simulink library "DAEMOT_Lib"  (R2019b)
settings: Solver=ode45  StartTime=0.0  StopTime=10.0  FixedStep=0.1  RelTol=1e-3
undefined symbols (not defined in the file or in its folder): Controller, CP, Ctrl, Ctrl_Fcn, Elec1, f, F2, Fluid, lag1, Mission, Moody, PropellerProp, rev_comms_sink
libraries: $bdroot x200, instrumentlib x21, simulink x5, dspsigops x2
(part 3 of 13)

== system DAEMOT_Lib/Legacy Components ==
  Aircraft : Subsystem  mask(Fluid Tank){Vel_init=300, M_dry=108500, M_load=21337, rho=0.243, A=360, Cd=0.02439}
      mask prompts: Vel_init "Initial Velocity [m/s]"; M_dry "Dry Weight [kg]"; M_load "Payload Weight [kg]"; rho "Air Density [kg/m^3]"; A "Reference Area [m²]"; Cd "Drag Coefficient [-]"
      mask help: Tracks the time rate of change for fluid mass and temperature.
      settings: OpenFcn=|
      | load('Fluids.mat');
      | Set_Fluid_Popup_Names( Fluid )
      mask DialogControl Container8 Prompt: Parameters
      mask Display:
      | image(imread('aircraft.jpg'))
      | 
      | text(0.5,0.9,['{\bf Aircraft}'],'TexMode','on','horizontalAlignment', 'center')
      | 
      | port_label('input',1,'Fuel Mass [kg]')
      | port_label('output',1,'Right Engine')
      | port_label('output',2,'Left Engine')
  Battery : Subsystem  mask{SOC0=0, C=100, P_max=100, T0=20, eta_max=0.98, T_max=100, eta_min=0.8}
      mask prompts: SOC0 "Initial State of Charge [0:1]"; C "Capacitance [MJ]"; P_max "Maximum Power [kW]"; T0 "Maximum Efficiency Temperature [oC]"; eta_max "Maximum Efficiency [0:1]"; T_max "Maximum Temperature [oC]"; eta_min "Minimum Efficiency [0:1]"
      mask init:
      | a = -(eta_max-eta_min)/(T_max-T0)^2;
      | b = -2*a*T0;
      | c = eta_max + a*T0^2;
      mask Display:
      | % text(0.5,0.9,['{\bf Load}'],'TexMode','on','horizontalAlignment', 'center')
      | 
      | port_label('input',1,'Power')
      | port_label('input',2,'Usage')
      | port_label('output',1,'Heat')
  Bus : Subsystem  mask(Bus){}
      mask help: This is a bus.
  Bus1 : Subsystem  mask(Bus){Num_Out=2}
      mask prompts: Num_Out "Number of Outputs"
      mask help: This is a bus.
      mask init:
      | h      = get_param(gcb,'handle');   % Get block handle
      | blk    = gcb;
      | hblock = get(h);     % Parse out handles structure
      | 
      | %%%%%%%%%%%%%%%%%%%%%%%%%%%%%% Clear Stuff %%%%%%%%%%%%%%%%%%%%%%%%%%%%%%%%
      | % delete any previous inports and bus selectors
      | for i = str2num(hblock.Num_Out)+1:hblock.Ports(2)
      |     delete_block([blk,'/Out',num2str(i)])
      |     delete_block([blk,'/b',num2str(i)])
      |     delete_block([blk,'/Source',num2str(i)])
      |     
      |     delete_unconnected_lines(blk)
      | end
      | %%%%%%%%%%%%%%%%%%%%%%%%%%%%%% Clear Stuff %%%%%%%%%%%%%%%%%%%%%%%%%%%%%%%%
      | 
      | %%%%%%%%%%%%%%%%%%%%%%%%%%%%%% Edit Mux inputs %%%%%%%%%%%%%%%%%%%%%%%%%%%%%%%%
      | 
      | set_param([blk,'/Add'],'Inputs',hblock.Num_Out)
      | 
      | %%%%%%%%%%%%%%%%%%%%%%%%%%%%%% Edit Mux inputs %%%%%%%%%%%%%%%%%%%%%%%%%%%%%%%%
      | 
      | %%%%%%%%%%%%%%%%%%%%%%%%%%%%%% Creat and Place Outputs %%%%%%%%%%%%%%%%%%%%%%%%%%%%%%%%
      | % generate outports, bus selectors, and route lines to each vector concat
      | for i = hblock.Ports(2)+1:str2num(hblock.Num_Out)
      |     
      |     % add blocks
      |     add_block('simulink/Ports & Subsystems/Out1',   [blk,'/Out',num2str(i)],   'Position',[900 i*80-25-180 900+30 i*80-12-180]);         % adding outport
      |     add_block('simulink/Signal Routing/Bus Creator',[blk,'/b',num2str(i)],     'Position',[850 i*80-20+20-218 850+5 i*80-2+20-198]);     % adding bus
      |     add_block('DAEMOT_Lib/Support Functions/Source', [blk,'/Source',num2str(i)],'Position',[400 i*80-205 400+65 i*80-180]);         % adding source
      | 
      |     % set bus number of ports
      |     set_param([blk,'/b',num2str(i)],'Inputs','2')
      |     
      | %     % set goto and from background colors
      | %     set_param([blk,'/t',num2str(i)],'BackgroundColor','cyan')
      | %     set_param([blk,'/m',num2str(i)],'BackgroundColor','cyan')
      | %     set_param([blk,'/p',num2str(i)],'BackgroundColor','cyan')
      | %     set_param([blk,'/g',num2str(i)],'BackgroundColor','cyan')
      | %     set_param([blk,'/mout',num2str(i)],'BackgroundColor','cyan')
      | %     %set_param([blk,'/tout',num2str(i)],'BackgroundColor','cyan')
      |     
      |     % add lines
      |     add_line(blk,['in/1'],['b',num2str(i),'/1'],'AutoRouting','on')
      |     
      |     add_line(blk,['Source',num2str(i),'/1'],['b',num2str(i),'/2'],'AutoRouting','on')
      |     p = get_param([blk,'/Source',num2str(i)],'PortHandles');
      |     l = get_param(p.Outport,'Line');
      |     set_param(l,'Name','I')
      |      
      |     add_line(blk,['b',num2str(i),'/1'],['Out',num2str(i),'/1'],'AutoRouting','on')
      |     add_line(blk,['Source',num2str(i),'/1'],['Add/',num2str(i)],'AutoRouting','on')
      | end
      | %%%%%%%%%%%%%%%%%%%%%%%%%%%%%% Create and Place Outputs %%%%%%%%%%%%%%%%%%%%%%%%%%%%%%%%
      | 
      | % try
      | %     set_param([blk,'/Selector1'],'InputPortWidth',num2str(hblock.Num_Out))
      | %     
      | %     selector_str = '[1 ';
      | %     for i = 2:str2num(hblock.Num_Out)
      | %         selector_str = [selector_str,num2str(i),' '];
      | %     end
      | %     selector_str = [selector_str,']'];
      | %     set_param([blk,'/Selector1'],'IndexParamArray',{selector_str})%num2cell(1:hblock.Num_Out))
      | % catch
      | %     selector_str = '[1 ';
      | %     for i = 2:str2num(hblock.Num_Out)
      | %         selector_str = [selector_str,num2str(i),' '];
      | %     end
      | %     selector_str = [selector_str,']'];
      | %     set_param([blk,'/Selector1'],'IndexParamArray',{selector_str})%num2cell(1:hblock.Num_Out))
      | %     
      | %     set_param([blk,'/Selector1'],'InputPortWidth',num2str(hblock.Num_Out))
      | % end 
      |     
      |     clear h blk hblock
      settings: CopyFcn=|
      | h      = get_param(gcb,'handle');   % Get block handle
      | blk    = gcb;
      | 
      | set_param(blk, 'LinkStatus', 'inactive')
      mask DialogControl ParameterTabVar0 Prompt: Bus Parameters
  Cabin : Subsystem  Commented=on  mask(Air Volume (Cabin)){T_init=0, V=0}
      mask prompts: T_init "Initial Temperature [°C]"; V "Volume [m³]"
      mask help: Tracks the time rate of change for the volume's temperature.
      mask init:
      | load Fluids
      | eval(['Fluid = Fluid.Air;']);
      mask DialogControl Container4 Prompt: Parameters
      mask Display:
      | text(0.5,0.95,['{\bf Air Volume}'],'TexMode','on','horizontalAlignment', 'center')
      | 
      | port_label('input',1,['Flow In'])
      | port_label('input',2,['Heat'])
      | port_label('output',1,['Flow Out'])
  Condenser : Subsystem  Commented=on  mask(Condenser){fld2=Water, T_init=0, C_wall=0, Tw0=0, Q0=0, T0=0, Tin_0=0, Tout_0=0, Qout_0=0, mdot2_0=0, H2_0=0, Tin2_0=0, A2=NaN, Rwc=NaN, Rc_in=NaN, Rc_out=NaN}
      mask prompts: fld2 "Secondary Fluid"; T_init "Initial Wall Temperature [°C]"; C_wall "Wall Capacitance [J/K]"; Tw0 "Condenser Wall Temperature [°C]"; Q0 "Wall Heat Transfer Rate [W]"; T0 "Condensing Temperature [°C]"; Tin_0 "Inlet Temperature [°C]"; Tout_0 "Outlet Temperature [°C]"; Qout_0 "Outlet Heat Transfer Rate [W]"; mdot2_0 "Mass Flow Rate [kg/s]"; H2_0 "Heat Transfer Coefficient [W/m²K]"; Tin2_0 "Fluid Inlet Temperature[°C]"; A2 "Heat Transfer Area [m²]"; Rwc "Condenser Wall Resistance"; Rc_in "Condenser Inlet Resistance"; Rc_out "Condenser Outlet Resistance"
      mask help: Tracks the time rate of change of condenser wall temperature. Calculates the outlet temperature and inlet/outlet heat flow.
      mask init:
      | load Fluids
      | eval(['F2 = Fluid.',get_param(gcb,'fld2'),';']);
      | 
      | 
      | area = -(mdot2_0*F2.cp/H2_0)*log(1-Q0/(mdot2_0*F2.cp*(Tw0 - Tin2_0)));    % m^2
      | 
      | Rwc = (T0 - Tw0) / Q0;
      | Rc_in = (Tin_0 - T0) / (Q0 - Qout_0);
      | Rc_out = (T0 - Tout_0)/(Qout_0);
      | 
      | set_param(gcb,'A2',num2str(area))
      | set_param(gcb,'Rwc',num2str(Rwc))
      | set_param(gcb,'Rc_in',num2str(Rc_in))
      | set_param(gcb,'Rc_out',num2str(Rc_out))
      mask TypeOptions fld2: Water | Fuel | Air
      mask DialogControl Container4 Prompt: Parameters
      mask DialogControl Container5 Prompt: Nonlinear Modeling
      mask DialogControl Container9 Prompt: Component Sizing - Nominal Values
      mask DialogControl Container10 Prompt: Primary Side
      mask DialogControl Container11 Prompt: Secondary Side
      mask DialogControl Container6 Prompt: Linear Model
      mask Display:
      | text(0.5,0.95,['{\bf Condenser}'],'TexMode','on','horizontalAlignment', 'center')
      | 
      | port_label('input',1,'Sink In')
      | port_label('input',2,'From Comp.')
      | port_label('input',3,'Inlet Resistance')
      | port_label('output',2,'To Valve')
      | port_label('output',1,'Sink Out')
  Converter : Subsystem  mask(Fluid Tank){V=230, I0=100, eta_max=0.98, eta_min=0.8}
      mask prompts: V "Converter Voltage [V]"; I0 "Maximum Efficiency Current [A]"; eta_max "Maximum Efficiency [0:1]"; eta_min "Minimum Efficiency [0:1]"
      mask help: Tracks the time rate of change for fluid mass and temperature.
      settings: OpenFcn=|
      | load('Fluids.mat');
      | Set_Fluid_Popup_Names( Fluid )
      mask DialogControl Container9 Prompt: Converter Parameters
      mask Display:
      | % image(imread('inverter.jpg'))
      | 
      | text(0.5,0.9,['{\bf Inverter}'],'TexMode','on','horizontalAlignment', 'center')
      | 
      | port_label('input',1,'In')
      | port_label('output',1,'Out')
      | port_label('output',2,'Heat')
  Dist : Subsystem  mask(Dist){}
      mask help: This is a distribution bus.
  Dist1 : Subsystem  mask{Num_In=2}
      mask prompts: Num_In "Number of Inputs"
      mask init:
      | h      = get_param(gcb,'handle');   % Get block handle
      | blk    = gcb;
      | hblock = get(h);     % Parse out handles structure
      | 
      | %%%%%%%%%%%%%%%%%%%%%%%%%%%%%% Clear Stuff %%%%%%%%%%%%%%%%%%%%%%%%%%%%%%%%
      | % delete any previous inports and bus selectors
      | for i = str2num(hblock.Num_In)+1:hblock.Ports(1)-1
      |     delete_block([blk,'/In',num2str(i)])
      |     delete_block([blk,'/b',num2str(i)])
      |     delete_block([blk,'/term',num2str(i)])
      |     delete_block([blk,'/Sink',num2str(i)])
      |     
      |     delete_unconnected_lines(blk)
      | end
      | if str2num(hblock.Num_In)+1 < hblock.Ports(1)-1
      | try
      | delete_block([blk,'/u'])
      | delete_unconnected_lines(blk)
      | end
      | end
      | %%%%%%%%%%%%%%%%%%%%%%%%%%%%%% Clear Stuff %%%%%%%%%%%%%%%%%%%%%%%%%%%%%%%%
      | 
      | %%%%%%%%%%%%%%%%%%%%%%%%%%%%%% Edit Mux inputs %%%%%%%%%%%%%%%%%%%%%%%%%%%%%%%%
      | set_param([blk,'/Mux'],'Inputs',hblock.Num_In)
      | set_param([blk,'/Demux'],'Outputs',hblock.Num_In)
      | %%%%%%%%%%%%%%%%%%%%%%%%%%%%%% Edit Mux inputs %%%%%%%%%%%%%%%%%%%%%%%%%%%%%%%%
      | 
      | %%%%%%%%%%%%%%%%%%%%%%%%%%%%%% Create and Place Inputs %%%%%%%%%%%%%%%%%%%%%%%%%%%%%%%%
      | % generate inports, bus selectors, and route lines to each vector concat
      | for i = hblock.Ports(1):str2num(hblock.Num_In)
      |     
      |     % add blocks
      |     add_block('simulink/Ports & Subsystems/In1',     [blk,'/In',num2str(i)],    'Position',[220 i*80+308 250 i*80+322]);         % adding inport
      |     add_block([blk,'/b1'],                           [blk,'/b',num2str(i)],    'Position',[295 i*80+275 300 i*80+355]);         % adding bus selector
      |     add_block('simulink/Sinks/Terminator',           [blk,'/term',num2str(i)],  'Position',[350 i*80+325 370 i*80+345]);         % adding terminator
      |     add_block('DAEMOT_Lib/Support Functions/Sink',   [blk,'/Sink',num2str(i)],  'Position',[1020 i*20+439 1085 i*20+461]);         % adding sink
      |     
      |     
      |     % set goto and from background colors
      | %    set_param([blk,'/gm',num2str(i)],'BackgroundColor','yellow')
      | %    set_param([blk,'/gt',num2str(i)],'BackgroundColor','yellow')
      | %    %set_param([blk,'/gp',num2str(i)],'BackgroundColor','yellow')
      | %    set_param([blk,'/min',num2str(i)],'BackgroundColor','yellow')
      | %    set_param([blk,'/tin',num2str(i)],'BackgroundColor','yellow')
      | %    set_param([blk,'/pout',num2str(i)],'BackgroundColor','cyan')
      |     
      |     % add lines
      |     add_line(blk,['In',num2str(i),'/1'], ['b',num2str(i),'/1'],'AutoRouting','on')
      |     add_line(blk,['b',num2str(i),'/1'], ['Mux/',num2str(i)],'AutoRouting','on')
      |     add_line(blk,['b',num2str(i),'/2'], ['term',num2str(i),'/1'],'AutoRouting','on')
      |     add_line(blk,['Demux/',num2str(i)], ['Sink',num2str(i),'/1'],'AutoRouting','on')
      |     
      | end
      | try
      |     add_block('simulink/Ports & Subsystems/In1',     [blk,'/u'],    'Position',[635-50 386+15 635-20 400+15]);         % adding control inport
      |     add_line(blk,['u/1'], ['u_tag/1'],'AutoRouting','on')
      | end
      | %%%%%%%%%%%%%%%%%%%%%%%%%%%%%% Creat and Place Inputs %%%%%%%%%%%%%%%%%%%%%%%%%%%%%%%%
      | 
      | % try
      | %     set_param([blk,'/Selector1'],'InputPortWidth',num2str(hblock.Num_In))
      | %     
      | %     selector_str = '[1 ';
      | %     for i = 2:str2num(hblock.Num_In)
      | %         selector_str = [selector_str,num2str(i),' '];
      | %     end
      | %     selector_str = [selector_str,']'];
      | %     set_param([blk,'/Selector1'],'IndexParamArray',{selector_str})%num2cell(1:hblock.Num_In))
      | % catch
      | %     selector_str = '[1 ';
      | %     for i = 2:str2num(hblock.Num_In)
      | %         selector_str = [selector_str,num2str(i),' '];
      | %     end
      | %     selector_str = [selector_str,']'];
      | %     set_param([blk,'/Selector1'],'IndexParamArray',{selector_str})%num2cell(1:hblock.Num_In))
      | %     
      | %     set_param([blk,'/Selector1'],'InputPortWidth',num2str(hblock.Num_In))
      | % end 
      |     
      |     clear h blk hblock
      settings: CopyFcn=|
      | h      = get_param(gcb,'handle');   % Get block handle
      | blk    = gcb;
      | 
      | set_param(blk, 'LinkStatus', 'inactive')
      mask DialogControl ParameterTabVar0 Prompt: Bus Parameters
  Engine : Subsystem  mask(Fluid Tank){fuel=Fuel, P=3500, Omega_init=1000, J=100, Omega_max=1500, Thrust_max=100000, eta=0.25, alpha=0.15}
      mask prompts: fuel "Fuel Type"; P "Engine Pressure [kPa]"; Omega_init "Initial Shaft Speed [rad/s]"; J "Moment of Inertia [kg m²]"; Omega_max "Maximum Shaft Speed [rad/s]"; Thrust_max "Maximum Thrust [N]"; eta "Engine Efficiency [-]"; alpha "Bearing Heat Gen Coeff. [kW/rad/s]"
      mask help: Tracks the time rate of change for fluid mass and temperature.
      mask init:
      | load('Fluids.mat');
      | Fuel = eval(['Fluid.',fuel]);
      settings: OpenFcn=|
      | load('Fluids.mat');
      | Set_Fluid_Popup_Names( Fluid )
      mask TypeOptions fuel: Fuel | Water | Air | PG50
      mask DialogControl Container9 Prompt: Engine Parameters
      mask Display:
      | image(imread('engine.jpg'))
      | 
      | text(0.5,0.9,['{\bf Engine}'],'TexMode','on','horizontalAlignment', 'center')
      | text(0.5,0.1,['{(P)}'],'TexMode','on','horizontalAlignment', 'center')
      | 
      | port_label('input',1,'Aircraft')
      | port_label('input',2,'Fuel In')
      | port_label('output',1,'Generator')
      | port_label('output',2,'Heat')
  Evaporator : Subsystem  Commented=on  mask(Evaporator){src=Heat Source (Q), fld=Fuel, T_init=0, C_wall=0, Tw0=0, Q0=0, T_evap=0, Tin_0=0, Tout_0=0, H0=0, Qin0=0, Qout0=0, mdot2_0=0, T2in_0=0, H2_0=0, A2=0, Rwe=NaN, Re_in=NaN, Re_out=NaN}
      mask prompts: src "Secondary Side Source"; fld "Fluid Type"; T_init "Initial Wall Temperature [°C]"; C_wall "Wall Capacitance [J/K]"; Tw0 "Evaporator Wall Temperature [°C]"; Q0 "Wall Heat Transfer Rate [W]"; T_evap "Evaporation Temperature [°C]"; Tin_0 "Inlet Temperature [°C]"; Tout_0 "Outlet Temperature [°C]"; H0 "Heat Transfer Coefficient [W/m²K]"; Qin0 "Inlet Heat Transfer Rate [W]"; Qout0 "Outlet Heat Transfer Rate [W]"; mdot2_0 "Mass Flow Rate [kg/s]"; T2in_0 "Inlet Temperature [°C]"; H2_0 "Heat Transfer Coefficient [W/m²K]"; A2 "Evaporator Wall Area [m²]"; Rwe "Evaporator Wall Resistance"; Re_in "Evaporator Inlet Resistance"; Re_out "Evaporator Outlet Resistance"
      mask help: Tracks the time rate of change of evaporator wall temperature. Calculates the outlet temperature and inlet/outlet heat flow.
      mask init:
      | load Fluids
      | eval(['F2 = Fluid.',get_param(gcb,'fld'),';']);
      | 
      | 
      | Rwe = (Tw0 - T_evap) / Q0;
      | Re_in = (Tin_0 - T_evap) / (Qin0);
      | Re_out = (T_evap - Tout_0) / (Qout0);
      | 
      | set_param(gcb,'Rwe',num2str(Rwe))
      | set_param(gcb,'Re_in',num2str(Re_in))
      | set_param(gcb,'Re_out',num2str(Re_out))
      | 
      | area = -((mdot2_0)*F2.cp/(H2_0+eps))*log(1-Q0/(mdot2_0*F2.cp*(T2in_0-Tw0)+eps));    % m^2
      |           
      | set_param(gcb,'A2',num2str(area))
      | 
      | 
      | % choices available in the popup menu
      | choices = {'Fluid Flow (Fluid Bus)','Heat Source (Q)'};
      | % index of the current choice
      | ndex = find(strcmp(get_param(gcb,'src'),choices));
      | 
      | if ndex == 1    % if fluid flow bus is selected
      |     try
      |         delete_line(gcb,'In2/1','Q_load_goto/1')
      |         delete_line(gcb,'In1/1','Tin_Bus/1')
      |         add_line(gcb,'In2/1','Tin_Bus/1')
      |     catch
      |     end
      |     set_param([gcb,'/outgain1'],'Gain','1')
      |     set_param([gcb,'/outgain2'],'Gain','1')
      | else            % if it is a heat source 
      |     try
      |         delete_line(gcb,'In2/1','Tin_Bus/1')
      |         add_line(gcb,'In2/1','Q_load_goto/1')
      |         add_line(gcb,'In1/1','Tin_Bus/1')
      |     catch
      |     end
      |     set_param([gcb,'/outgain1'],'Gain','0')
      |     set_param([gcb,'/outgain2'],'Gain','0')
      | end
      | 
      | clear ndex choices
      mask TypeOptions src: Fluid Flow (Fluid Bus) | Heat Source (Q)
      mask Callback src:
      | % choices available in the popup menu
      | choices = {'Fluid Flow (Fluid Bus)','Heat Source (Q)'};
      | % index of the current choice
      | ndex = find(strcmp(get_param(gcb,'src'),choices));
      | % visibility of parameters in the mask
      | mask_vis = get_param(gcb,'MaskVisibilities');
      | 
      | % maskobj = Simulink.Mask.get(gcb);
      | % dialogobj = maskobj.getDialogControls();
      | % grpobj = dialogobj(1, 2).DialogControls(1, 2).DialogControls.DialogControls(1, 5);
      | 
      | if ndex == 1    % if fluid flow bus is selected
      |     mask_vis{2} = 'on';    mask_vis{13} = 'on';    mask_vis{14} = 'on';
      |     mask_vis{15} = 'on';    mask_vis{16} = 'on';
      | 
      | else            % if it is a heat source
      |     mask_vis{2} = 'off';    mask_vis{13} = 'off';    mask_vis{14} = 'off';
      |     mask_vis{15} = 'off';    mask_vis{16} = 'off';
      | 
      | end
      | 
      | % setting the new visibility
      | set_param(gcb,'MaskVisibilities',mask_vis)
      | 
      | clear ndex choices mask_vis maskobj dialogobj grpobj
      mask TypeOptions fld: Fuel | Water | Air
      mask DialogControl Container4 Prompt: Parameters
      mask DialogControl Container5 Prompt: Nonlinear Model
      mask DialogControl Container7 Prompt: Component Sizing - Nominal Values
      mask DialogControl Container9 Prompt: Primary Side
      mask DialogControl SecSideContainer Prompt: Secondary Side
      mask DialogControl Container6 Prompt: Linear Model
      mask Display:
      | text(0.5,0.95,['{\bf Evaporator}'],'TexMode','on','horizontalAlignment', 'center')
      | 
      | port_label('input',1,'From Valve')
      | % choices available in the popup menu
      | choices = {'Fluid Flow (Fluid Bus)','Heat Source (Q)'};
      | % index of the current choice
      | ndex = find(strcmp(get_param(gcb,'src'),choices));
      | 
      | if ndex == 1
      |     port_label('input',2,'Secondary Flow')
      |     port_label('output',2,'Secondary Flow')
      | elseif ndex == 2
      |     port_label('input',2,'Heat Source (Q)')
      |     port_label('output',2,'<null>')
      | else
      |     port_label('input',2,'ERROR IN MASK')
      | end
      | 
      | port_label('input',3,'Outlet Resistance')
      | port_label('output',1,'To Comp.')
  Fan : Subsystem  mask(Liquid Pump){P_init=145, T_init=22, D=13*1e-3, L=0.1, rho=1000, cp=4, E=0, Omega_max=3000, DP_max=20, mdot_max=0.5, alpha=0.001}
      mask prompts: P_init "Intial Outlet Pressure [kPa]"; T_init "Intial Outlet Temperature [°C]"; D "Pipe Internal Diameter [m]"; L "Pipe Length [m]"; rho "Air Density [kg/m^3]"; cp "Air Specific Heat [kJ/kgK]"; E "Air Modulus of Elasticity [N/m^2]"; Omega_max "Maximum Shaft Speed [RPM]"; DP_max "Maximum Pressure Difference [kPa]"; mdot_max "Maximum Mass Flow Rate [kg/s]"; alpha "Heat Generation Coefficient [kW/RPM]"
      mask help: Tracks the time rate of change of fluid temperature, mass flow rate, and power consumption.
      mask init:
      | load('Fluids.mat');
      | Fluid = eval(['Fluid.Air']);
      settings: OpenFcn=|
      | load('Fluids.mat');
      | Set_Fluid_Popup_Names( Fluid )
      mask DialogControl Container11 Prompt: Parameters
      mask DialogControl Container14 Prompt: Nonlinear Model
      mask DialogControl Container15 Prompt: Component Sizing - Nominal Values
      mask Display:
      | % image(imread('centpump.jpg'))
      | 
      | text(0.5,0.95,['{\bf Fan}'],'TexMode','on','horizontalAlignment', 'center')
      | text(0.5,0.1,['{-----(P)}'],'TexMode','on','horizontalAlignment', 'center')
      | 
      | port_label('input',1,'Flow In')
      | port_label('input',2,'Power')
      | port_label('input',3,'Shaft Speed [RPM]')
      | port_label('output',1,'Flow Out')
  Fan1 : Subsystem  Commented=on  mask(Fan){fld=Air, T_init=0, tau=10, alpha=0.002, beta=0, lambda=3e-4, gamma=00, k=0, omega0=1000, Power0=300, mdot0=2, lin_mdl=on, T0=0, P0=0}
      mask prompts: fld "Fluid Type"; T_init "Intial Fluid Temperature [°C]"; tau "Time Constant (tau)"; omega0 "Rotational Speed [RPM]"; Power0 "Power [W]"; mdot0 "Mass Flow Rate [kg/s]"; lin_mdl "Enable Linear Model"; T0 "Temperature [°C]"; P0 "Power [W]"
      mask help: Tracks the time rate of change of fluid temperature, mass flow rate, and power consumption.
      mask init:
      | % A = [-1/tau];
      | % B = 0;
      | % V = [1/tau];
      | % 
      | % C = [1; 0; 0];
      | % D = [0; alpha; 2*lambda*omega0+gamma];
      | % W = [0; 0; 0];
      | 
      | mdot = alpha*omega0+beta;  % kg/s
      | set_param(gcb,'mdot0',num2str(mdot));
      | 
      | Power = lambda*omega0^2+gamma*omega0+k;    % W
      | set_param(gcb,'Power0',num2str(Power));
      mask TypeOptions fld: Fuel | Water | Air
      mask DialogControl Control2 Prompt: dT/dt = (Tin-T)/tau
      mask DialogControl Control3 Prompt: dm/dt = alpha*omega+beta
      mask DialogControl Control4 Prompt: P=gamma*omega^2 + gamma*omega + k
      mask DialogControl Container11 Prompt: Parameters
      mask DialogControl Container14 Prompt: Nonlinear Model
      mask DialogControl Container8 Prompt: Pump Model
      mask DialogControl Container5 Prompt: Power Consumption Model
      mask DialogControl Container15 Prompt: Nominal Values
      mask DialogControl Container17 Prompt: Linear Model
      mask DialogControl Container4 Prompt: Linearization Point
      mask Display:
      | text(0.5,0.95,['{\bf Fan}'],'TexMode','on','horizontalAlignment', 'center')
      | 
      | port_label('input',1,'Flow In')
      | port_label('input',2,'Speed [RPM]')
      | port_label('output',1,'Flow Out')
  Flow Flow Source (Pressure) : Subsystem  mask(Flow Source (Pressure)){M_ext=on, M=0, T_ext=on, T=0, P_ext=on, P=0}
      mask prompts: M_ext "Mass flow rate time varying?"; M "Mass flow rate (kg/s)"; T_ext "Temperature time varying?"; T "Temperature (C)"; P_ext "Pressure time varying?"; P "Pressure (kPa)"
      mask help: Used to create a flow source.
      mask Callback M_ext:
      | en = get_param(gcb,'MaskVisibilities');
      | h      = get_param(gcb,'handle');   % Get block handle
      | blk    = gcb;
      | hblock = get(h);     % Parse out handles structure
      | 
      | switch get_param(gcb,'M_ext')
      |     case 'on'
      |         en{2} = 'off';
      |         %add_block('simulink/Ports & Subsystems/In1',   [blk,'/In1'],'Position',[130    -7   160     7]);         % adding inport
      | 
      |     case 'off'
      |         en{2} = 'on';
      |         %delete_block([blk,'/In1'])
      | 
      | end
      | set_param(gcb,'MaskVisibilities',en);
      mask Callback T_ext:
      | en = get_param(gcb,'MaskVisibilities');
      | 
      | switch get_param(gcb,'T_ext')
      |     case 'on'
      |         en{4} = 'off';
      |     case 'off'
      |         en{4} = 'on';
      | end
      | set_param(gcb,'MaskVisibilities',en);
      mask Callback P_ext:
      | en = get_param(gcb,'MaskVisibilities');
      | 
      | switch get_param(gcb,'P_ext')
      |     case 'on'
      |         en{6} = 'off';
      |     case 'off'
      |         en{6} = 'on';
      | end
      | set_param(gcb,'MaskVisibilities',en);
      mask Display:
      | text(0.5,0.95,['{\bf Pressure Source}'],'TexMode','on','horizontalAlignment', 'center')
      | text(0.5,0.1,['{(start)}'],'TexMode','on','horizontalAlignment', 'center')
      | 
      | port_label('input',1,'Source Temperature (C)')
      | port_label('input',2,'Source Pressure (kPa)')
      | 
      | port_label('output',1,'Source')
  Flow Sink (Mass Flow Rate) : Subsystem  mask(Flow Sink (Mass Flow Rate)){M_ext=on, M=0, T_ext=on, T=0, P_ext=on, P=0}
      mask prompts: M_ext "Mass flow rate time varying?"; M "Mass flow rate (kg/s)"; T_ext "Temperature time varying?"; T "Temperature (C)"; P_ext "Pressure time varying?"; P "Pressure (kPa)"
      mask help: Used to create a flow sink.
      mask Callback M_ext:
      | en = get_param(gcb,'MaskVisibilities');
      | h      = get_param(gcb,'handle');   % Get block handle
      | blk    = gcb;
      | hblock = get(h);     % Parse out handles structure
      | 
      | switch get_param(gcb,'M_ext')
      |     case 'on'
      |         en{2} = 'off';
      |         %add_block('simulink/Ports & Subsystems/In1',   [blk,'/In1'],'Position',[130    -7   160     7]);         % adding inport
      | 
      |     case 'off'
      |         en{2} = 'on';
      |         %delete_block([blk,'/In1'])
      | 
      | end
      | set_param(gcb,'MaskVisibilities',en);
      mask Callback T_ext:
      | en = get_param(gcb,'MaskVisibilities');
      | 
      | switch get_param(gcb,'T_ext')
      |     case 'on'
      |         en{4} = 'off';
      |     case 'off'
      |         en{4} = 'on';
      | end
      | set_param(gcb,'MaskVisibilities',en);
      mask Callback P_ext:
      | en = get_param(gcb,'MaskVisibilities');
      | 
      | switch get_param(gcb,'P_ext')
      |     case 'on'
      |         en{6} = 'off';
      |     case 'off'
      |         en{6} = 'on';
      | end
      | set_param(gcb,'MaskVisibilities',en);
      mask Display:
      | text(0.5,0.95,['{\bf Mass Flow Rate Sink}'],'TexMode','on','horizontalAlignment', 'center')
      | text(0.5,0.1,['{-----end}'],'TexMode','on','horizontalAlignment', 'center')
      | 
      | port_label('input',1,'Sink')
      | port_label('input',2,'Sink Mass Flow Rate (kg/s)')
  Flow Sink (Pressure) : Subsystem  mask(Flow Sink (Pressure)){M_ext=on, M=0, T_ext=on, T=0, P_ext=on, P=0}
      mask prompts: M_ext "Mass flow rate time varying?"; M "Mass flow rate (kg/s)"; T_ext "Temperature time varying?"; T "Temperature (C)"; P_ext "Pressure time varying?"; P "Pressure (kPa)"
      mask help: Used to create a flow sink.
      mask Callback M_ext:
      | en = get_param(gcb,'MaskVisibilities');
      | h      = get_param(gcb,'handle');   % Get block handle
      | blk    = gcb;
      | hblock = get(h);     % Parse out handles structure
      | 
      | switch get_param(gcb,'M_ext')
      |     case 'on'
      |         en{2} = 'off';
      |         %add_block('simulink/Ports & Subsystems/In1',   [blk,'/In1'],'Position',[130    -7   160     7]);         % adding inport
      | 
      |     case 'off'
      |         en{2} = 'on';
      |         %delete_block([blk,'/In1'])
      | 
      | end
      | set_param(gcb,'MaskVisibilities',en);
      mask Callback T_ext:
      | en = get_param(gcb,'MaskVisibilities');
      | 
      | switch get_param(gcb,'T_ext')
      |     case 'on'
      |         en{4} = 'off';
      |     case 'off'
      |         en{4} = 'on';
      | end
      | set_param(gcb,'MaskVisibilities',en);
      mask Callback P_ext:
      | en = get_param(gcb,'MaskVisibilities');
      | 
      | switch get_param(gcb,'P_ext')
      |     case 'on'
      |         en{6} = 'off';
      |     case 'off'
      |         en{6} = 'on';
      | end
      | set_param(gcb,'MaskVisibilities',en);
      mask Display:
      | text(0.5,0.95,['{\bf Pressure Sink}'],'TexMode','on','horizontalAlignment', 'center')
      | text(0.5,0.1,['{(end)}'],'TexMode','on','horizontalAlignment', 'center')
      | 
      | port_label('input',1,'Sink')
      | port_label('input',2,'Sink Pressure (kPa)')
  Flow Source (Mass Flow Rate) : Subsystem  mask(Flow Source (Mass Flow Rate)){M_ext=on, M=0, T_ext=on, T=0, P_ext=on, P=0}
      mask prompts: M_ext "Mass flow rate time varying?"; M "Mass flow rate (kg/s)"; T_ext "Temperature time varying?"; T "Temperature (C)"; P_ext "Pressure time varying?"; P "Pressure (kPa)"
      mask help: Used to create a flow source.
      mask Callback M_ext:
      | en = get_param(gcb,'MaskVisibilities');
      | h      = get_param(gcb,'handle');   % Get block handle
      | blk    = gcb;
      | hblock = get(h);     % Parse out handles structure
      | 
      | switch get_param(gcb,'M_ext')
      |     case 'on'
      |         en{2} = 'off';
      |         %add_block('simulink/Ports & Subsystems/In1',   [blk,'/In1'],'Position',[130    -7   160     7]);         % adding inport
      | 
      |     case 'off'
      |         en{2} = 'on';
      |         %delete_block([blk,'/In1'])
      | 
      | end
      | set_param(gcb,'MaskVisibilities',en);
      mask Callback T_ext:
      | en = get_param(gcb,'MaskVisibilities');
      | 
      | switch get_param(gcb,'T_ext')
      |     case 'on'
      |         en{4} = 'off';
      |     case 'off'
      |         en{4} = 'on';
      | end
      | set_param(gcb,'MaskVisibilities',en);
      mask Callback P_ext:
      | en = get_param(gcb,'MaskVisibilities');
      | 
      | switch get_param(gcb,'P_ext')
      |     case 'on'
      |         en{6} = 'off';
      |     case 'off'
      |         en{6} = 'on';
      | end
      | set_param(gcb,'MaskVisibilities',en);
      mask Display:
      | text(0.5,0.95,['{\bf Mass Flow Rate Source}'],'TexMode','on','horizontalAlignment', 'center')
      | text(0.5,0.1,['{start-----}'],'TexMode','on','horizontalAlignment', 'center')
      | 
      | port_label('input',1,'Source Temperature (C)')
      | port_label('input',2,'Source Mass Flow Rate (kg/s)')
      | 
      | port_label('output',1,'Source')
  Flow Split_Junction_Wall : Subsystem  AncestorBlock=DAEMOT_Lib/Components/Flow Split_Junction  mask(Split/Junction with Wall){fld=PG50, Num_Out=1, Num_In=1, P_init=200, T_init=30, Tw_init=22, f=0.05, A_ht=0.1, PAF=1, HTC_method=off, HTC=1000, D=0.013, L=0.1, t=0.0015, E=2.4e6, v=0.4, M_wall=1, Cp_wall=0.9}
      mask prompts: fld "Fluid Type"; Num_Out "Number of Outlet Flows"; Num_In "Number of Inlet Flows"; P_init "Initial Pressure [kPa]"; T_init "Initial Temperature [°C]"; Tw_init "Initial Wall Temperature [°C]"; f "Friction Factor [-]"; A_ht "Heat Transfer Area [m^2]"; PAF "HTC Parameter Adjustment Factor [-]"; HTC_method "User-Defined Heat Transfer Coefficient?"; HTC "Heat Transfer Coefficient [W/m^2*K]"; D "Diameter [m]"; L "Length [m]"; t "Tube Wall Thickness [m]"; E "Tube Modulus of Elasticity [kPa]"; v "Tube Poisson Ratio [-]"; M_wall "Wall Mass [kg]"; Cp_wall "Wall Specific Heat [kJ/kg*K]"
      mask help: Splits and junctions flows using dynamic relationships. Also models convective heat transfer with a wall to which an exogenous heat load is applied. Note that the library link of the block is disabled when it is imported into a model.
      mask init:
      | h      = get_param(gcb,'handle');   % Get block handle
      | blk    = gcb;
      | hblock = get(h);     % Parse out handles structure
      | 
      | load('Fluids.mat');
      | Fluid = eval(['Fluid.',fld]);
      | 
      | 
      | try
      |     delete_line(blk,['In',num2str(hblock.Ports(1)),'/1'],'Q_BUS/1')
      | catch
      | end
      | 
      | % delete any previous inports and bus selectors
      | for i = str2num(hblock.Num_In)+1:hblock.Ports(1)-1
      |     delete_block([blk,'/gb',num2str(i)])
      |     delete_block([blk,'/gm',num2str(i)])
      |     delete_block([blk,'/gt',num2str(i)])
      |     delete_block([blk,'/gp',num2str(i)])
      |     delete_block([blk,'/Sink',num2str(i)])
      |     delete_block([blk,'/pout',num2str(i)])
      |     delete_block([blk,'/min',num2str(i)])
      |     delete_block([blk,'/tin',num2str(i)])
      |     
      |     delete_unconnected_lines(blk)
      | end
      | for i = str2num(hblock.Num_In)+2:hblock.Ports(1)-1
      |     delete_block([blk,'/In',num2str(i)])
      | end
      | for i=str2num(hblock.Num_In)+2:hblock.Ports(1)
      |     try
      |         delete_block([blk,'/In',num2str(i)])
      |     catch
      |     end
      | end
      | 
      | % delete any previous inports and bus selectors
      | for i = str2num(hblock.Num_Out)+1:hblock.Ports(2)
      |     delete_block([blk,'/Out',num2str(i)])
      |     delete_block([blk,'/m',num2str(i)])
      |     delete_block([blk,'/t',num2str(i)])
      |     delete_block([blk,'/p',num2str(i)])
      |     delete_block([blk,'/b',num2str(i)])
      |     delete_block([blk,'/Source',num2str(i)])
      |     delete_block([blk,'/g',num2str(i)])
      |     delete_block([blk,'/mout',num2str(i)])
      |     %delete_block([blk,'/tout',num2str(i)])
      |     
      |     delete_unconnected_lines(blk)
      | end
      | 
      | set_param([blk,'/Mux_In_1'],'Inputs',hblock.Num_In)
      | set_param([blk,'/Mux_In_2'],'Inputs',hblock.Num_Out)
      | set_param([blk,'/Mux_In_3'],'Inputs',hblock.Num_In)
      | 
      | % generate inports, bus selectors, and route lines to each vector concat
      | for i = hblock.Ports(1):str2num(hblock.Num_In)
      |     
      |     % add blocks
      |     try
      |         add_block('simulink/Ports & Subsystems/In1',   [blk,'/In',num2str(i)],    'Position',[120 i*80-25+20 150 i*80-12+20]);         % adding inport
      |     catch
      |     end
      |     add_block([blk,'/gb1'],                        [blk,'/gb',num2str(i)],   'Position',[200 i*80-20+20-18 205 i*80-2+20+2]);         % adding inport
      |     add_block('simulink/Signal Routing/Goto',      [blk,'/gm',num2str(i)],    'Position',[260 i*80-17 340 i*80-3]);         % adding inport
      |     add_block('simulink/Signal Routing/Goto',      [blk,'/gt',num2str(i)],    'Position',[260 i*80+3 340 i*80+17]);         % adding inport
      |     add_block('simulink/Sinks/Terminator',          [blk,'/gp',num2str(i)],    'Position',[260 i*80+23 280 i*80+37]);         % adding inport
      |     add_block('DAEMOT_Lib/Support Functions/Sink',[blk,'/Sink',num2str(i)],'Position',[745 i*80-14 810 i*80+14]);         % adding inport
      |     add_block('simulink/Signal Routing/From',      [blk,'/pout',num2str(i)],    'Position',[625 i*80-14 705 i*80+14]);         % adding inport
      |     add_block('simulink/Signal Routing/From',       [blk,'/min',num2str(i)],     'Position',[935 -258+i*20 1015 -242+i*20]);         % adding inport
      |     add_block('simulink/Signal Routing/From',       [blk,'/tin',num2str(i)],     'Position',[935 1+i*20 1015 19+i*20]);         % adding inport
      |     
      |     % set goto and from tags
      |     set_param([blk,'/gm',num2str(i)],'GotoTag',char(horzcat('M_in',num2str(i))))
      |     set_param([blk,'/gt',num2str(i)],'GotoTag',char(horzcat('T_in',num2str(i))))
      |     %set_param([blk,'/gp',num2str(i)],'GotoTag',char(horzcat('P_in',num2str(i))))
      |     set_param([blk,'/pout',num2str(i)],'GotoTag',char('P'))
      |     set_param([blk,'/min',num2str(i)],'GotoTag',char(horzcat('M_in',num2str(i))))
      |     set_param([blk,'/tin',num2str(i)],'GotoTag',char(horzcat('T_in',num2str(i))))
      |     
      |     % set goto and from background colors
      |     set_param([blk,'/gm',num2str(i)],'BackgroundColor','yellow')
      |     set_param([blk,'/gt',num2str(i)],'BackgroundColor','yellow')
      |     %set_param([blk,'/gp',num2str(i)],'BackgroundColor','yellow')
      |     set_param([blk,'/min',num2str(i)],'BackgroundColor','yellow')
      |     set_param([blk,'/tin',num2str(i)],'BackgroundColor','yellow')
      |     set_param([blk,'/pout',num2str(i)],'BackgroundColor','cyan')
      |     
      |     % add lines
      |     add_line(blk,['In',num2str(i),'/1'], ['gb',num2str(i),'/1'],'AutoRouting','on')
      |     add_line(blk,['gb',num2str(i),'/1'],  ['gm',num2str(i),'/1'],'AutoRouting','on')
      |     add_line(blk,['gb',num2str(i),'/2'],  ['gt',num2str(i),'/1'],'AutoRouting','on')
      |     add_line(blk,['gb',num2str(i),'/3'],  ['gp',num2str(i),'/1'],'AutoRouting','on')
      |     add_line(blk,['pout',num2str(i),'/1'],  ['Sink',num2str(i),'/1'],'AutoRouting','on')
      |     add_line(blk,['min',num2str(i),'/1'],  ['Mux_In_1/',num2str(i)],'AutoRouting','on')
      |     add_line(blk,['tin',num2str(i),'/1'],  ['Mux_In_3/',num2str(i)],'AutoRouting','on')
      |     
      | end
      | 
      | % generate inports, bus selectors, and route lines to each vector concat
      | for i = hblock.Ports(2)+1:str2num(hblock.Num_Out)
      |     
      |     % add blocks
      |     add_block('simulink/Ports & Subsystems/Out1',   [blk,'/Out',num2str(i)],   'Position',[30 i*80-25+20 60 i*80-12+20]);         % adding inport
      |     add_block('simulink/Signal Routing/From',       [blk,'/m',num2str(i)],     'Position',[-150 i*80-20 -70 i*80-2]);         % adding inport
      |     add_block('simulink/Signal Routing/From',       [blk,'/t',num2str(i)],     'Position',[-150 i*80-20+20 -70 i*80-2+20]);         % adding inport
      |     add_block('simulink/Signal Routing/From',       [blk,'/p',num2str(i)],     'Position',[-150 i*80-20+40 -70 i*80-2+40]);         % adding inport
      |     add_block('simulink/Signal Routing/Bus Creator',[blk,'/b',num2str(i)],     'Position',[5 i*80-20+20-18 10 i*80-2+20+2]);         % adding inport
      |     add_block('DAEMOT_Lib/Support Functions/Source',[blk,'/Source',num2str(i)],'Position',[395 i*80-14 460 i*80+14]);         % adding inport
      |     add_block('simulink/Signal Routing/Goto',       [blk,'/g',num2str(i)],     'Position',[505 i*80-9 585 i*80+9]);         % adding inport
      |     add_block('simulink/Signal Routing/From',       [blk,'/mout',num2str(i)],  'Position',[935 -129+i*20 1015 -111+i*20]);         % adding inport
      |     %add_block('simulink/Signal Routing/Goto',      [blk,'/tout',num2str(i)],   'Position',[1455 -259+i*20 1535 -241+i*20]);         % adding inport
      |     
      |     % set goto and from tags
      |     set_param([blk,'/m',num2str(i)],'GotoTag',char(horzcat('M_out',num2str(i))))
      |     %set_param([blk,'/t',num2str(i)],'GotoTag',char(horzcat('T_out',num2str(i))))
      |     set_param([blk,'/t',num2str(i)],'GotoTag',char('T'))
      |     set_param([blk,'/p',num2str(i)],'GotoTag',char('P'))
      |     set_param([blk,'/g',num2str(i)],'GotoTag',char(horzcat('M_out',num2str(i))))
      |     set_param([blk,'/mout',num2str(i)],'GotoTag',char(horzcat('M_out',num2str(i))))
      |     %set_param([blk,'/tout',num2str(i)],'GotoTag',char(horzcat('T_out',num2str(i))))
      |     set_param([blk,'/b',num2str(i)],'Inputs','3')
      |     
      |     % set goto and from background colors
      |     set_param([blk,'/t',num2str(i)],'BackgroundColor','cyan')
      |     set_param([blk,'/m',num2str(i)],'BackgroundColor','cyan')
      |     set_param([blk,'/p',num2str(i)],'BackgroundColor','cyan')
      |     set_param([blk,'/g',num2str(i)],'BackgroundColor','cyan')
      |     set_param([blk,'/mout',num2str(i)],'BackgroundColor','cyan')
      |     %set_param([blk,'/tout',num2str(i)],'BackgroundColor','cyan')
      |     
      |     % add lines
      |     add_line(blk,['m',num2str(i),'/1'],['b',num2str(i),'/1'],'AutoRouting','on')
      |     p = get_param([blk,'/m',num2str(i)],'PortHandles');
      |     l = get_param(p.Outport,'Line');
      |     set_param(l,'Name','mdot_kgps')
      |     
      |     add_line(blk,['t',num2str(i),'/1'],['b',num2str(i),'/2'],'AutoRouting','on')
      |     p = get_param([blk,'/t',num2str(i)],'PortHandles');
      |     l = get_param(p.Outport,'Line');
      |     set_param(l,'Name','T_C')
      |     
      |     add_line(blk,['p',num2str(i),'/1'],['b',num2str(i),'/3'],'AutoRouting','on')
      |     p = get_param([blk,'/p',num2str(i)],'PortHandles');
      |     l = get_param(p.Outport,'Line');
      |     set_param(l,'Name','P_kPa')
      |     
      |     add_line(blk,['b',num2str(i),'/1'],['Out',num2str(i),'/1'],'AutoRouting','on')
      |     add_line(blk,['Source',num2str(i),'/1'],['g',num2str(i),'/1'],'AutoRouting','on')
      |     add_line(blk,['mout',num2str(i),'/1'],  ['Mux_In_2/',num2str(i)],'AutoRouting','on')
      |     %add_line(blk,['Mux_Out_1/',num2str(i)], ['tout',num2str(i),'/1'],'AutoRouting','on')
      | end
      | 
      | try
      |     set_param([blk,'/Selector1'],'InputPortWidth',num2str(hblock.Num_In))
      |     set_param([blk,'/Selector2'],'InputPortWidth',num2str(hblock.Num_In))
      |     
      |     selector_str = '[1 ';
      |     for i = 2:str2num(hblock.Num_In)
      |         selector_str = [selector_str,num2str(i),' '];
      |     end
      |     selector_str = [selector_str,']'];
      |     set_param([blk,'/Selector1'],'IndexParamArray',{selector_str})%num2cell(1:hblock.Num_In))
      |     set_param([blk,'/Selector2'],'IndexParamArray',{selector_str})%num2cell(1:hblock.Num_In))
      | catch
      |     selector_str = '[1 ';
      |     for i = 2:str2num(hblock.Num_In)
      |         selector_str = [selector_str,num2str(i),' '];
      |     end
      |     selector_str = [selector_str,']'];
      |     set_param([blk,'/Selector1'],'IndexParamArray',{selector_str})%num2cell(1:hblock.Num_In))
      |     set_param([blk,'/Selector2'],'IndexParamArray',{selector_str})%num2cell(1:hblock.Num_In))
      |     
      |     set_param([blk,'/Selector1'],'InputPortWidth',num2str(hblock.Num_In))
      |     set_param([blk,'/Selector2'],'InputPortWidth',num2str(hblock.Num_In))
      | end
      | 
      | try
      |     add_block('simulink/Ports & Subsystems/In1',   [blk,'/In',num2str(str2num(hblock.Num_In)+1)],    'Position',[120 80-25+20 150 80-12+20]);         % adding inport
      | catch
      | end
      | try
      |     add_line(blk,['In',num2str(str2num(hblock.Num_In)+1),'/1'],'Q_BUS/1','AutoRouting','on')
      | catch
      | end
      | 
      | clear h blk hblock
      settings: CopyFcn=|
      | h      = get_param(gcb,'handle');   % Get block handle
      | blk    = gcb;
      | 
      | set_param(blk, 'LinkStatus', 'inactive')
      settings: OpenFcn=|
      | load('Fluids.mat');
      | Set_Fluid_Popup_Names( Fluid )
      mask TypeOptions fld: Fuel | Water | Air | PG50
      mask Callback HTC_method:
      | en = get_param(gcb,'MaskVisibilities');
      | 
      | switch get_param(gcb,'HTC_method')
      |     case 'on'
      |         en{11} = 'on';
      |     case 'off'
      |         en{11} = 'off';
      | end
      | set_param(gcb,'MaskVisibilities',en);
      mask DialogControl Container4 Prompt: Parameters
      mask DialogControl Container12 Prompt: Nonlinear Model
      mask DialogControl Container15 Prompt: Component Sizing - Nominal Values
      mask Display:
      | image(imread('Split.jpg'));
      | 
      | text(0.5,0.95,['{\bf',fld,' Split/Junction with Wall}'],'TexMode','on','horizontalAlignment', 'center')
      | text(0.5,0.08,['{(P)}'],'TexMode','on','horizontalAlignment', 'center')
      | 
      | h      = get_param(gcb,'handle');   % Get block handle
      | blk    = gcb;
      | hblock = get(h);     % Parse out handles structure
      | for i = 1:str2num(hblock.Num_In)
      |     port_label('input',i,horzcat('Flow In #',num2str(i)))
      | end
      | for i = 1:str2num(hblock.Num_Out)
      |     port_label('output',i,horzcat('Flow Out #',num2str(i)))
      | end
      | port_label('input',str2num(hblock.Num_In)+1,'Heat Load [kW]')
  Fluid Tank : Subsystem  mask(Fluid Tank){fld=PG50, T_init=22, h_init=0.2, M_init=1.0433, P_init=103.0361, Tamb_init=22, H=0, D=0.08, Pamb=101}
      mask prompts: fld "Fluid Type"; T_init "Initial Fluid Temperature [°C]"; h_init "Initial Fluid Height [m]"; M_init "Initial Fluid Mass [kg] (fcn of height)"; P_init "Initial Fluid Pressure [kPa] (fcn of height)"; Tamb_init "Initial Ambient Temperature [°C]"; H "Heat Transfer Coefficient [W/m²K]"; D "Tank Diameter [m]"; Pamb "Ambient Pressure [kPa]"
      mask help: Tracks the time rate of change for fluid mass and temperature.
      mask init:
      | load('Fluids.mat');
      | Fluid = eval(['Fluid.',fld]);
      | 
      | % Note: Assumes a fixed initial pressure to calculate density
      | P_for_rho = 105;
      | Rho = qminterp2(Fluid.T, Fluid.P, Fluid.Rho_pt, T_init, P_for_rho);
      | 
      | M_init = h_init*Rho*pi*D^2/4;
      | set_param(gcb,'M_init',num2str(M_init));
      | 
      | P_init = Rho*9.81*h_init/1000 + Pamb;
      | set_param(gcb,'P_init',num2str(P_init));
      settings: OpenFcn=|
      | load('Fluids.mat');
      | Set_Fluid_Popup_Names( Fluid )
      mask TypeOptions fld: Fuel | Water | Air | PG50
      mask DialogControl Container8 Prompt: Parameters
      mask DialogControl Container10 Prompt: Nonlinear Model
      mask DialogControl NomValuesGroupVar Prompt: Component Sizing - Nominal Values
      mask DialogControl Container11 Prompt: Linear Model
      mask Display:
      | image(imread('Res.jpg'))
      | 
      | text(0.5,0.95,['{\bf ',fld,' Tank}'],'TexMode','on','horizontalAlignment', 'center')
      | text(0.5,0.08,['{(P)}'],'TexMode','on','horizontalAlignment', 'center')
      | 
      | port_label('input',1,'Flow In')
      | port_label('input',2,'Amb. Temp. [°C]')
      | port_label('output',1,'Flow Out')
  From LabVIEW_Old : Subsystem  Commented=on  mask(LabView Measurements){n_meas=46, config_loc=0}
      mask prompts: n_meas "Number of measurements from LabView"; config_loc "LabVIEW Config File Location (.json)"
      mask help: This block reads from the localhost across port 61556. Data is transmitted from LabVEW over the port. The bus names are taken from a configuration file generated within LabVIEW. The update rate is hard-coded to 10 Hz.
      mask init:
      | h = gcbh;
      | param = get(h);
      | blk = [param.Path, '/', param.Name,'/UDP Receive'];
      | h = get_param(blk,'handle');
      | 
      | set_param(h,'DataSize',['[',num2str(n_meas),' 1]'])
      mask Display:
      | if n_meas > 1
      |     port_label('output',1,['Mux - ',num2str(n_meas),' signals'])
      | else
      |     port_label('output',1,['Mux - ',num2str(n_meas),' signal'])
      | end
  Generator : Subsystem  mask(Fluid Tank){V=230, eta=0.98}
      mask prompts: V "Generator Voltage"; eta "Generator Efficiency"
      mask help: Tracks the time rate of change for fluid mass and temperature.
      settings: OpenFcn=|
      | load('Fluids.mat');
      | Set_Fluid_Popup_Names( Fluid )
      mask DialogControl Container9 Prompt: Generator Parameters
      mask Display:
      | image(imread('generator.jpg'))
      | 
      | text(0.5,0.9,['{\bf Generator}'],'TexMode','on','horizontalAlignment', 'center')
      | 
      | port_label('input',1,'Engine')
      | port_label('output',1,'Bus')
      | port_label('output',2,'Heat')
  Graph Sink : Subsystem  mask(Effort Sink (Torque)){Stype=Voltage Sink, const=on, value=0}
      mask prompts: Stype "Sink Type"; const "Constant Value?"; value "Voltage [V]"
      mask help: Used to create a effot sink.
      mask init: same as DAEMOT_Lib/Electrical/Effort Sink
      settings: CopyFcn=|
      | h      = get_param(gcb,'handle');   % Get block handle
      | blk    = gcb;
      | 
      | set_param(blk, 'LinkStatus', 'inactive')
      | clear h
      | clear blk
      mask TypeOptions Stype: Voltage Sink | Current Sink | Angular Speed Sink | Torque Sink | Temperature Sink | Heat Flow Sink
      mask Callback Stype:
      | mp = get_param(gcb,'MaskPrompts');
      | h      = get_param(gcb,'handle');   % Get block handle
      | blk    = gcb;
      | hblock = get(h);     % Parse out handles structure
      | 
      | switch get_param(gcb,'Stype')
      |     case 'Voltage Sink'
      |         mp{3} = 'Voltage [V]';
      |     case 'Current Sink'
      |         mp{3} = 'Current [A]';
      |     case 'Angular Speed Sink'
      |         mp{3} = 'Speed [rad/s]';
      |     case 'Torque Sink'
      |         mp{3} = 'Torque [Nm]';
      |     case 'Temperature Sink'
      |         mp{3} = 'Temperature [C]';
      |     case 'Heat Flow Sink'
      |         mp{3} = 'Heat Flow [kW]';
      | end
      | set_param(gcb,'MaskPrompts',mp);
      mask Callback const:
      | en = get_param(gcb,'MaskVisibilities');
      | h      = get_param(gcb,'handle');   % Get block handle
      | blk    = gcb;
      | hblock = get(h);     % Parse out handles structure
      | 
      | switch get_param(gcb,'const')
      |     case 'on'
      |         en{3} = 'on';
      | %         delete_block([blk,'/In1'])
      | 
      |     case 'off'
      |         en{3} = 'off';
      | %         add_block('simulink/Ports & Subsystems/In1',   [blk,'/In1'],'Position',[130    -7   160     7]);         % adding inport
      | 
      | end
      | set_param(gcb,'MaskVisibilities',en);
      | 
      | % hblock.MaskPrompts{3} = 'hello';
      mask Display:
      | text(0.45,0.90,['{\bf',get_param(gcb,'Stype'),'}'],'TexMode','on','horizontalAlignment', 'center')
      | % text(0.5,0.1,['{(T)(end)}'],'TexMode','on','horizontalAlignment', 'center')
      | 
      | type = get_param(gcb,'Stype');
      | switch type
      |         case 'Voltage Sink'
      |             nm = 'Voltage [V]';
      |             id = '(V)';
      |             un = 'V';
      |         case 'Current Sink'
      |             nm = 'Current [A]';
      |             id = '(----)';
      |             un = 'A';
      |         case 'Angular Speed Sink'
      |             nm = 'Speed [rad/s]';
      |             id = '(----)';
      |             un = 'rad/s';
      |         case 'Torque Sink'
      |             nm = 'Torque [Nm]';
      |             id = '(\tau)';
      |             un = 'Nm';
      |         case 'Temperature Sink'
      |             nm = 'Temperature [C]';
      |             id = '(T)';
      |             un = 'C';
      |         case 'Heat Flow Sink'
      |             nm = 'Heat Flow [kW]';
      |             id = '(----)';
      |             un = 'kW';
      | end
      | 
      | if strcmp(get_param(gcb,'const'),'on')
      |     text(0.75,0.500,['{\bf',get_param(gcb,'Value'),un,'}'],'TexMode','on','horizontalAlignment', 'center')
      | else
      |     port_label('input',2,sprintf(['Sink ',nm]));
      | end
      | 
      | 
      | port_label('input',1,'Sink');
      | text(0.5,0.175,['{',id,' (end)}'],'TexMode','on','horizontalAlignment', 'center');
  Graph Source : Subsystem  mask(Effort Source (Voltage)){Stype=Voltage Source, const=on, value=0}
      mask prompts: Stype "Source Type"; const "Constant Value?"; value "Voltage [V]"
      mask help: Used to create an effort source.
      mask init: same as DAEMOT_Lib/Electrical/Effort Source
      settings: CopyFcn=|
      | h      = get_param(gcb,'handle');   % Get block handle
      | blk    = gcb;
      | 
      | set_param(blk, 'LinkStatus', 'inactive')
      | clear h
      | clear blk
      mask TypeOptions Stype: Voltage Source | Current Source | Angular Speed Source | Torque Source | Temperature Source | Heat Flow Source
      mask Callback Stype:
      | mp = get_param(gcb,'MaskPrompts');
      | h      = get_param(gcb,'handle');   % Get block handle
      | blk    = gcb;
      | hblock = get(h);     % Parse out handles structure
      | 
      | switch get_param(gcb,'Stype')
      |     case 'Voltage Source'
      |         mp{3} = 'Voltage [V]';
      |     case 'Current Source'
      |         mp{3} = 'Current [A]';
      |     case 'Angular Speed Source'
      |         mp{3} = 'Speed [rad/s]';
      |     case 'Torque Source'
      |         mp{3} = 'Torque [Nm]';
      |     case 'Temperature Source'
      |         mp{3} = 'Temperature [C]';
      |     case 'Heat Flow Source'
      |         mp{3} = 'Heat Flow [kW]';
      | end
      | set_param(gcb,'MaskPrompts',mp);
      mask Callback const:
      | en = get_param(gcb,'MaskVisibilities');
      | h      = get_param(gcb,'handle');   % Get block handle
      | blk    = gcb;
      | hblock = get(h);     % Parse out handles structure
      | 
      | switch get_param(gcb,'const')
      |     case 'on'
      |         en{3} = 'on';
      | %         delete_block([blk,'/In1'])
      | 
      |     case 'off'
      |         en{3} = 'off';
      | %         add_block('simulink/Ports & Subsystems/In1',   [blk,'/In1'],'Position',[130    -7   160     7]);         % adding inport
      | 
      | end
      | set_param(gcb,'MaskVisibilities',en);
      | 
      | % hblock.MaskPrompts{3} = 'hello';
      mask Display:
      | text(0.45,0.900,['{\bf',get_param(gcb,'Stype'),'}'],'TexMode','on','horizontalAlignment', 'center')
      | 
      | type = get_param(gcb,'Stype');
      | switch type
      |         case 'Voltage Source'
      |             nm = 'Voltage [V]';
      |             id = '(V)*';
      |             un = 'V';
      |         case 'Current Source'
      |             nm = 'Current [A]';
      |             id = '(----)';
      |             un = 'A';
      |         case 'Angular Speed Source'
      |             nm = 'Speed [rad/s]';
      |             id = '(----)';
      |             un = 'rad/s';
      |         case 'Torque Source'
      |             nm = 'Torque [Nm]';
      |             id = '(\tau)*';
      |             un = 'Nm';
      |         case 'Temperature Source'
      |             nm = 'Temperature [C]';
      |             id = '(T)';
      |             un = 'C';
      |         case 'Heat Flow Source'
      |             nm = 'Heat Flow [kW]';
      |             id = '(----)';
      |             un = 'kW';
      | end
      | 
      | if strcmp(get_param(gcb,'const'),'on')
      |     text(0.25,0.500,['{\bf',get_param(gcb,'Value'),un,'}'],'TexMode','on','horizontalAlignment', 'center')
      | else
      |     port_label('input',1,sprintf(['Source \n',nm]))
      | end
      | port_label('output',1,'Source')
      | text(0.5,0.175,['{(start) ',id,'}'],'TexMode','on','horizontalAlignment', 'center')
  Heat Sink (Temp) : Subsystem  mask(Power Sink (Temp)){}
      mask help: Used to create a power sink.
      mask Display:
      | text(0.5,0.95,['{\bf Heat Sink}'],'TexMode','on','horizontalAlignment', 'center')
      | text(0.5,0.1,['{(end)}'],'TexMode','on','horizontalAlignment', 'center')
      | 
      | port_label('input',1,'Sink')
      | port_label('input',2,'Sink Temp (oC)')
  Heater : Subsystem  mask{P_max=100}
      mask prompts: P_max "Maximum Power [kW]"
      mask Display:
      | % text(0.5,0.9,['{\bf Load}'],'TexMode','on','horizontalAlignment', 'center')
      | 
      | port_label('input',1,'Power')
      | port_label('input',2,'Usage')
      | port_label('output',1,'Heat')
  LabVIEW_UDP_old : Subsystem  Commented=on  mask(LabView Measurements){n_in=48, n_out=0, config_loc=C:\Users\pangbor2\Desktop\Matlab.json}
      mask prompts: n_in "Number of measurements from LabView"; n_out "Number of measurements to LabView"; config_loc "LabVIEW Config File Location (.json)"
      mask help: This block sends data to and from LabVIEW over UDP. The bus names are taken from a configuration file generated within LabVIEW. The update rate is hard-coded to 10 Hz.
      mask init:
      | h      = get_param(gcb,'handle');   % Get block handle
      | blk    = gcb;
      | hblock = get(h);     % Parse out handles structure
      | 
      | % Load .json file
      | fname = config_loc;
      | fid = fopen(fname);
      | raw = fread(fid,inf);
      | str = char(raw');
      | fclose(fid);
      | val = jsondecode(str)
      | 
      | % Retrieve data of interest
      | signals_in = val{1,1}
      | signals_out = val{2,1}
      | 
      | % Remove empty cells
      | signals_in  = signals_in(~cellfun(@isempty,signals_in))
      | signals_out = signals_out(~cellfun(@isempty,signals_out))
      | 
      | % Create valid MATLAB varible names
      | signals_in  = matlab.lang.makeValidName(signals_in)
      | signals_out = matlab.lang.makeValidName(signals_out)
      | 
      | n_in  = length(signals_in)
      | n_out = length(signals_out)
      | 
      | % Set Demux and Bus Creator dimensions
      | set_param([blk,'/Demux'],'Outputs',num2str(n_in))
      | set_param([blk,'/Bus Creator'],'Inputs',num2str(n_in))
      | 
      | % Get line handles
      | p = get_param([blk,'/Demux'],'PortHandles')
      | l = get_param(p.Outport,'Line')
      | 
      | for i=1:n_in
      |     try
      |         % Draw lines
      |         add_line(blk,['Demux/',num2str(i)], ['Bus Creator/',num2str(i)],'AutoRouting','on')
      |     catch
      |         set_param(l{i},'Name',signals_in{i})
      |     end
      | end
      | 
      | delete_unconnected_lines(blk)
      | 
      | % Generate string of bus names to LabVIEW
      | out_str = '';
      | for i=1:n_out-1
      |     out_str = [out_str,[signals_out{i},',']];
      | end
      | out_str = [out_str,signals_out{n_out}];
      | 
      | set_param([blk,'/Bus Selector'],'OutputSignals',out_str)
      mask Display:
      | port_label('input',1,['Bus to LabVIEW - ',num2str(n_in),' signals'])
      | port_label('output',1,['Bus from LabVIEW - ',num2str(n_out),' signals'])
  Load : Subsystem  mask{P_max=100}
      mask prompts: P_max "Maximum Power [kW]"
      mask Display:
      | % text(0.5,0.9,['{\bf Load}'],'TexMode','on','horizontalAlignment', 'center')
      | 
      | port_label('input',1,'Power')
      | port_label('input',2,'Usage')
  MEMC_Comp : Subsystem  Commented=on  mask(MEMC Compressor){Tk_in_init=0, Tk_out_init=0, eta=0, Ck_in=0, Ck_out=0, alpha=0, beta=0, k=0, gamma=0}
      mask prompts: Tk_in_init "Initial Inlet Temperature [°C]"; Tk_out_init "Initial Outlet Temperature [°C]"; eta "Compressor Efficiency [%]"; Ck_in "Inlet Capacitance"; Ck_out "Outlet Capacitance"; gamma "Power Coefficients [a1 a2 a3 a4]"
      mask help: Tracks the time rate of change of the inlet and exit temperatures of the refrigerant. Calculates power consumption.
      mask DialogControl Container4 Prompt: Parameters
      mask DialogControl Container5 Prompt: Nonlinear Model
      mask DialogControl Control3 Prompt: Q = omega*(alpha*Tout + beta*Tin + k)
      mask DialogControl Container7 Prompt: Power Consumption Model
      mask DialogControl Control4 Prompt: P=(omega^2 + a1*omega)*(a2*Tout + a3*Tin + a4)
      mask DialogControl Container6 Prompt: Linear Model
      mask Display:
      | text(0.5,0.95,['{\bf MEMC Comp.}'],'TexMode','on','horizontalAlignment', 'center')
      | 
      | port_label('input',1,'Evap1')
      | port_label('input',2,'Evap2')
      | port_label('input',3,'Evap3')
      | port_label('input',4,'Evap4')
      | port_label('input',5,'Speed [RPM]')
      | port_label('output',1,'Cond1')
      | port_label('output',2,'Cond2')
  MEMC_Valves : Subsystem  Commented=on  mask(MEMC Valve){T_init=0, Cv=1}
      mask prompts: T_init "Initial Temperature [°C]"; Cv "Valve Capacitance [J/K]"
      mask help: Tracks the time rate of change of the exit flow temperature.
      mask DialogControl Container4 Prompt: Parameters
      mask DialogControl Container5 Prompt: Nonlinear Model
      mask DialogControl Container8 Prompt: Linear Model
      mask Display:
      | text(0.5,0.95,['{\bf MEMC Valves}'],'TexMode','on','horizontalAlignment', 'center')
      | 
      | port_label('input',1,'Cond1')
      | port_label('input',2,'Cond2')
      | port_label('output',1,'Evap1')
      | port_label('output',2,'Evap2')
      | port_label('output',3,'Evap3')
      | port_label('output',4,'Evap4')
  Pipe_M_to_M : Subsystem  Commented=on  mask(Pipe (M to M)){fld=PG50, Tout_init=22, P_init=110, Tamb_init=22, H=0, D=13*1e-3, L=0.2, e=0.01*1e-3}
      mask prompts: fld "Fluid Type"; Tout_init "Initial Outlet Temperature [°C]"; P_init "Initial Fluid Pressure [kPa]"; Tamb_init "Initial Ambient Temperature [°C]"; H "Heat Transfer Coefficient [W/m²K]"; D "Pipe Internal Diameter [m]"; L "Pipe Length [m]"; e "Surface Roughness [m] (0.0015mm for copper, 0.01mm for rubber, 0mm for plastic)"
      mask help: Models a pipe given upstream and downstream mass flow rates.
      mask init:
      | load('Fluids.mat');
      | Fluid = eval(['Fluid.',fld]);
      | 
      | load('Moody.mat');
      settings: OpenFcn=|
      | load('Fluids.mat');
      | Set_Fluid_Popup_Names( Fluid )
      mask TypeOptions fld: Fuel | Water | Air | PG50
      mask DialogControl Container8 Prompt: Parameters
      mask DialogControl Container10 Prompt: Nonlinear Model
      mask DialogControl NomValuesGroupVar Prompt: Component Sizing - Nominal Values
      mask DialogControl Container11 Prompt: Linear Model
      mask Display:
      | image(imread('Tube.jpg'))
      | 
      | text(0.5,0.95,['{\bf ',fld,' Pipe (M to M)}'],'TexMode','on','horizontalAlignment', 'center')
      | text(0.5,0.1,['{(P)}'],'TexMode','on','horizontalAlignment', 'center')
      | 
      | port_label('input',1,'Flow In')
      | port_label('input',2,'Amb. Temp. [°C]')
      | port_label('output',1,'Flow Out')
  Pipe_M_to_P : Subsystem  Commented=on  mask(Pipe (M to P)){fld=PG50, Tout_init=22, P_init=149.9, Tamb_init=22, H=0, D=13*1e-3, L=0.2, e=0.01*1e-3}
      mask prompts: fld "Fluid Type"; Tout_init "Initial Outlet Temperature [°C]"; P_init "Initial Inlet Pressure [kPa]"; Tamb_init "Initial Ambient Temperature [°C]"; H "Heat Transfer Coefficient [W/m²K]"; D "Pipe Internal Diameter [m]"; L "Pipe Length [m]"; e "Surface Roughness [m] (0.0015mm for copper, 0.01mm for rubber, 0mm for plastic)"
      mask help: Models a pipe given an upstream mass flow rate and downstream pressure.
      mask init:
      | load('Fluids.mat');
      | Fluid = eval(['Fluid.',fld]);
      | 
      | load('Moody.mat');
      settings: OpenFcn=|
      | load('Fluids.mat');
      | Set_Fluid_Popup_Names( Fluid )
      mask TypeOptions fld: Fuel | Water | Air | PG50
      mask DialogControl Container8 Prompt: Parameters
      mask DialogControl Container10 Prompt: Nonlinear Model
      mask DialogControl NomValuesGroupVar Prompt: Component Sizing - Nominal Values
      mask DialogControl Container11 Prompt: Linear Model
      mask Display:
      | image(imread('Tube.jpg'))
      | 
      | text(0.5,0.95,['{\bf ',fld,' Pipe (M to P)}'],'TexMode','on','horizontalAlignment', 'center')
      | text(0.5,0.1,['{(P)-----}'],'TexMode','on','horizontalAlignment', 'center')
      | 
      | port_label('input',1,'Flow In')
      | port_label('input',2,'Amb. Temp. [°C]')
      | port_label('output',1,'Flow Out')
  Pipe_P_to_M1 : Subsystem  Commented=on  mask(Sensor/Valve (P to M)){fld=PG50, Comp_Type=Pressure Sensor, T_init=22, P_init=101, Tamb_init=22, f=0.05, KL=0, H=0, D=13*1e-3, L=0.1, t=0.0015, E=2.4e6, v=0.4, dH=0, e_rough=0.01*1e-3}
      mask prompts: fld "Fluid Type"; Comp_Type "Sensor/Valve Type"; T_init "Initial Outlet Temperature [°C]"; P_init "Initial Outlet Pressure [kPa]"; Tamb_init "Initial Ambient Temperature [°C]"; f "Friction Factor [-]"; KL "Minor Losses [-]"; H "Heat Transfer Coefficient [W/m²K]"; D "Pipe Internal Diameter [m]"; L "Length [m]"; t "Tube Wall Thickness [m]"; E "Tube Modulus of Elasticity [kPa]"; v "Tube Poisson Ratio [-]"; dH "Height between Inlet and Outlet [m]"; e_rough "Surface Roughness [m] (0.0015mm for copper, 0.01mm for rubber, 0mm for plastic)"
      mask help: Models a sensor or valve given an upstream pressure and downstream mass flow rate.
      mask init:
      | load('Fluids.mat');
      | Fluid = eval(['Fluid.',fld]);
      | 
      | load('Moody.mat');
      settings: OpenFcn=|
      | load('Fluids.mat');
      | Set_Fluid_Popup_Names( Fluid )
      mask TypeOptions fld: Fuel | Water | Air | PG50
      mask TypeOptions Comp_Type: Mass Flow Rate Sensor | Pressure Sensor | Temperature Sensor | Ball Valve | Check Valve
      mask DialogControl Container8 Prompt: Parameters
      mask DialogControl Container10 Prompt: Nonlinear Model
      mask DialogControl NomValuesGroupVar Prompt: Component Sizing - Nominal Values
      mask DialogControl Container11 Prompt: Linear Model
      mask Display:
      | if Comp_Type <=3
      |     image(imread('Sensor.jpg'))
      | else
      |     image(imread('Valve.jpg'))
      | end
      | 
      | text(0.5,0.95,['{\bf ',fld,' Sensor/Valve (P to M)}'],'TexMode','on','horizontalAlignment', 'center')
      | text(0.5,0.1,['{-----(P)}'],'TexMode','on','horizontalAlignment', 'center')
      | 
      | port_label('input',1,'Flow In')
      | port_label('output',1,'Flow Out')
  Pipe_P_to_M_Wall : Subsystem  mask(Pipe with Wall Convection (P to M)){fld=PG50, T_init=20, P_init=101, Tamb_init=22, f=0.05, KL_tube=0, KL=0, A_ht=0.1, PAF=1, HTC_method=on, HTC=4000, H=0, D=13*1e-3, L=0.1, t=0.0015, E=2.4e6, v=0.4, dH=0, e_rough=0.01*1e-3, Num_MFRS=0, Num_PS=0, Num_TS=0, Num_BV=0, Num_CV=0}
      mask prompts: fld "Fluid Type"; T_init "Initial Outlet Temperature [°C]"; P_init "Initial Outlet Pressure [kPa]"; Tamb_init "Initial Ambient Temperature [°C]"; f "Tube Friction Factor [-]"; KL_tube "Tube Minor Losses [-]"; KL "Total Minor Losses [-]"; A_ht "Heat Transfer Area [m^2]"; PAF "HTC Parameter Adjustment Factor [-]"; HTC_method "User-Defined Heat Transfer Coefficient?"; HTC "Heat Transfer Coefficient [W/m^2*K]"; H "Heat Transfer Coefficient [W/m²K]"; D "Pipe Internal Diameter [m]"; L "Pipe Length [m]"; t "Tube Wall Thickness [m]"; E "Tube Modulus of Elasticity [kPa]"; v "Tube Poisson Ratio [-]"; dH "Height between Inlet and Outlet [m]"; e_rough "Surface Roughness [m] (0.0015mm for copper, 0.01mm for rubber, 0mm for plastic)"; Num_MFRS "Number of Mass Flow Rate Sensors"; Num_PS "Number of Pressure Sensors"; Num_TS "Number of Temperature Sensors"; Num_BV "Number of Ball Valves"; Num_CV "Number of Check Valves"
      mask help: Models a pipe given an upstream pressure and downstream mass flow rate. Also models convective heat transfer to a separate wall block.
      mask init:
      | load('Fluids.mat');
      | Fluid = eval(['Fluid.',fld]);
      | 
      | load('Moody.mat');
      | 
      | KL = KL_correction(KL_tube,Num_MFRS,Num_PS,Num_TS,Num_BV,Num_CV);
      | set_param(gcb,'KL',num2str(KL));
      settings: OpenFcn=|
      | load('Fluids.mat');
      | Set_Fluid_Popup_Names( Fluid )
      mask TypeOptions fld: Fuel | Water | Air | PG50
      mask Callback HTC_method:
      | en = get_param(gcb,'MaskVisibilities');
      | 
      | switch get_param(gcb,'HTC_method')
      |     case 'on'
      |         en{11} = 'on';
      |     case 'off'
      |         en{11} = 'off';
      | end
      | set_param(gcb,'MaskVisibilities',en);
      mask DialogControl Container8 Prompt: Parameters
      mask DialogControl Container10 Prompt: Nonlinear Model
      mask DialogControl NomValuesGroupVar Prompt: Component Sizing - Nominal Values
      mask DialogControl Container11 Prompt: Linear Model
      mask DialogControl Container16 Prompt: Sensors and Valves
      mask Display:
      | if sum([Num_MFRS,Num_PS,Num_TS,Num_BV,Num_CV])==0
      |     image(imread('Tube.jpg'))
      | elseif sum([Num_MFRS,Num_PS,Num_TS])~=0 && sum([Num_BV,Num_CV])==0
      |     image(imread('Tube_Sensor.jpg'))
      | elseif sum([Num_MFRS,Num_PS,Num_TS])==0 && sum([Num_BV,Num_CV])~=0
      |     image(imread('Tube_Valve.jpg'))
      | else
      |     image(imread('Tube_Valve_Sensor.jpg'))
      | end
      | 
      | text(0.5,0.95,['{\bf ',fld,' Pipe with Wall Convection (P to M)}'],'TexMode','on','horizontalAlignment', 'center')
      | text(0.5,0.1,['{-----(P)}'],'TexMode','on','horizontalAlignment', 'center')
      | 
      | port_label('input',1,'Flow In')
      | port_label('input',2,'Wall')
      | port_label('output',1,'Flow Out')
  Pipe_P_to_M_with_Heat_Load : Subsystem  mask(Pipe with Heat Load (P to M)){fld=PG50, T_init=22, P_init=101, Tamb_init=22, f=0.05, KL_tube=0, KL=0, H=0, D=13*1e-3, L=0.1, t=0.0015, E=2.4e6, v=0.4, dH=0, e_rough=0.01*1e-3, Num_MFRS=0, Num_PS=0, Num_TS=0, Num_BV=0, Num_CV=0}
      mask prompts: fld "Fluid Type"; T_init "Initial Outlet Temperature [°C]"; P_init "Initial Outlet Pressure [kPa]"; Tamb_init "Initial Ambient Temperature [°C]"; f "Tube Friction Factor [-]"; KL_tube "Tube Minor Losses [-]"; KL "Total Minor Losses [-]"; H "Heat Transfer Coefficient [W/m²K]"; D "Pipe Internal Diameter [m]"; L "Pipe Length [m]"; t "Tube Wall Thickness [m]"; E "Tube Modulus of Elasticity [kPa]"; v "Tube Poisson Ratio [-]"; dH "Height between Inlet and Outlet [m]"; e_rough "Surface Roughness [m] (0.0015mm for copper, 0.01mm for rubber, 0mm for plastic)"; Num_MFRS "Number of Mass Flow Rate Sensors"; Num_PS "Number of Pressure Sensors"; Num_TS "Number of Temperature Sensors"; Num_BV "Number of Ball Valves"; Num_CV "Number of Check Valves"
      mask help: Models a pipe given an upstream pressure and downstream mass flow rate. Also models a heat load applied to the fluid.
      mask init:
      | load('Fluids.mat');
      | Fluid = eval(['Fluid.',fld]);
      | 
      | load('Moody.mat');
      | 
      | KL = KL_correction(KL_tube,Num_MFRS,Num_PS,Num_TS,Num_BV,Num_CV);
      | set_param(gcb,'KL',num2str(KL));
      settings: OpenFcn=|
      | load('Fluids.mat');
      | Set_Fluid_Popup_Names( Fluid )
      mask TypeOptions fld: Fuel | Water | Air | PG50
      mask DialogControl Container8 Prompt: Parameters
      mask DialogControl Container10 Prompt: Nonlinear Model
      mask DialogControl NomValuesGroupVar Prompt: Component Sizing - Nominal Values
      mask DialogControl Container11 Prompt: Linear Model
      mask DialogControl Container16 Prompt: Sensors and Valves
      mask Display:
      | if sum([Num_MFRS,Num_PS,Num_TS,Num_BV,Num_CV])==0
      |     image(imread('Tube.jpg'))
      | elseif sum([Num_MFRS,Num_PS,Num_TS])~=0 && sum([Num_BV,Num_CV])==0
      |     image(imread('Tube_Sensor.jpg'))
      | elseif sum([Num_MFRS,Num_PS,Num_TS])==0 && sum([Num_BV,Num_CV])~=0
      |     image(imread('Tube_Valve.jpg'))
      | else
      |     image(imread('Tube_Valve_Sensor.jpg'))
      | end
      | 
      | text(0.5,0.95,['{\bf ',fld,' Pipe with Heat Load (P to M)}'],'TexMode','on','horizontalAlignment', 'center')
      | text(0.5,0.1,['{-----(P)}'],'TexMode','on','horizontalAlignment', 'center')
      | 
      | port_label('input',1,'Flow In')
      | port_label('input',2,'Heat Load [kW]')
      | port_label('output',1,'Flow Out')
  Pipe_P_to_P1 : Subsystem  Commented=on  mask(Sensor/Valve (P to P)){fld=PG50, Comp_Type=Mass Flow Rate Sensor, T_init=22, Tamb_init=22, f=0.05, KL=0, H=0, D=13*1e-3, L=0.1, t=0.0015, E=2.4e6, v=0.4, dH=0, e_rough=0.01*1e-3}
      mask prompts: fld "Fluid Type"; Comp_Type "Sensor/Valve Type"; T_init "Initial Outlet Temperature [°C]"; Tamb_init "Initial Ambient Temperature [°C]"; f "Friction Factor [-]"; KL "Minor Losses [-]"; H "Heat Transfer Coefficient [W/m²K]"; D "Internal Diameter [m]"; L "Length [m]"; t "Tube Wall Thickness [m]"; E "Tube Modulus of Elasticity [kPa]"; v "Tube Poisson Ratio [-]"; dH "Height between Inlet and Outlet [m]"; e_rough "Surface Roughness [m] (0.0015mm for copper, 0.01mm for rubber, 0mm for plastic)"
      mask help: Models a sensor or valve given upstream and downstream pressures.
      mask init:
      | load('Fluids.mat');
      | Fluid = eval(['Fluid.',fld]);
      | 
      | load('Moody.mat');
      settings: OpenFcn=|
      | load('Fluids.mat');
      | Set_Fluid_Popup_Names( Fluid )
      mask TypeOptions fld: Fuel | Water | Air | PG50
      mask TypeOptions Comp_Type: Mass Flow Rate Sensor | Pressure Sensor | Temperature Sensor | Ball Valve | Check Valve
      mask DialogControl Container8 Prompt: Parameters
      mask DialogControl Container10 Prompt: Nonlinear Model
      mask DialogControl NomValuesGroupVar Prompt: Component Sizing - Nominal Values
      mask DialogControl Container11 Prompt: Linear Model
      mask Display:
      | if Comp_Type <=3
      |     image(imread('Sensor.jpg'))
      | else
      |     image(imread('Valve.jpg'))
      | end
      | 
      | text(0.5,0.95,['{\bf ',fld,' Sensor/Valve (P to P)}'],'TexMode','on','horizontalAlignment', 'center')
      | text(0.5,0.1,['{-----}'],'TexMode','on','horizontalAlignment', 'center')
      | 
      | port_label('input',1,'Flow In')
      | port_label('output',1,'Flow Out')
  Power Sink (Current) : Subsystem  mask(Power Sink (Current)){M_ext=on, M=0, T_ext=on, T=0, P_ext=on, P=0}
      mask prompts: M_ext "Mass flow rate time varying?"; M "Mass flow rate (kg/s)"; T_ext "Temperature time varying?"; T "Temperature (C)"; P_ext "Pressure time varying?"; P "Pressure (kPa)"
      mask help: Used to create a power sink.
      mask Callback M_ext:
      | en = get_param(gcb,'MaskVisibilities');
      | h      = get_param(gcb,'handle');   % Get block handle
      | blk    = gcb;
      | hblock = get(h);     % Parse out handles structure
      | 
      | switch get_param(gcb,'M_ext')
      |     case 'on'
      |         en{2} = 'off';
      |         %add_block('simulink/Ports & Subsystems/In1',   [blk,'/In1'],'Position',[130    -7   160     7]);         % adding inport
      | 
      |     case 'off'
      |         en{2} = 'on';
      |         %delete_block([blk,'/In1'])
      | 
      | end
      | set_param(gcb,'MaskVisibilities',en);
      mask Callback T_ext:
      | en = get_param(gcb,'MaskVisibilities');
      | 
      | switch get_param(gcb,'T_ext')
      |     case 'on'
      |         en{4} = 'off';
      |     case 'off'
      |         en{4} = 'on';
      | end
      | set_param(gcb,'MaskVisibilities',en);
      mask Callback P_ext:
      | en = get_param(gcb,'MaskVisibilities');
      | 
      | switch get_param(gcb,'P_ext')
      |     case 'on'
      |         en{6} = 'off';
      |     case 'off'
      |         en{6} = 'on';
      | end
      | set_param(gcb,'MaskVisibilities',en);
      mask Display:
      | text(0.5,0.95,['{\bf Current Sink}'],'TexMode','on','horizontalAlignment', 'center')
      | text(0.5,0.1,['{(end)}'],'TexMode','on','horizontalAlignment', 'center')
      | 
      | port_label('input',1,'Sink')
      | port_label('input',2,'Sink Current (A)')
  Power Source (Voltage) : Subsystem  mask(Power Source (Voltage)){M_ext=on, M=0, T_ext=on, T=0, P_ext=on, P=0}
      mask prompts: M_ext "Mass flow rate time varying?"; M "Mass flow rate (kg/s)"; T_ext "Temperature time varying?"; T "Temperature (C)"; P_ext "Pressure time varying?"; P "Pressure (kPa)"
      mask help: Used to create a power source.
      mask Callback M_ext:
      | en = get_param(gcb,'MaskVisibilities');
      | h      = get_param(gcb,'handle');   % Get block handle
      | blk    = gcb;
      | hblock = get(h);     % Parse out handles structure
      | 
      | switch get_param(gcb,'M_ext')
      |     case 'on'
      |         en{2} = 'off';
      |         %add_block('simulink/Ports & Subsystems/In1',   [blk,'/In1'],'Position',[130    -7   160     7]);         % adding inport
      | 
      |     case 'off'
      |         en{2} = 'on';
      |         %delete_block([blk,'/In1'])
      | 
      | end
      | set_param(gcb,'MaskVisibilities',en);
      mask Callback T_ext:
      | en = get_param(gcb,'MaskVisibilities');
      | 
      | switch get_param(gcb,'T_ext')
      |     case 'on'
      |         en{4} = 'off';
      |     case 'off'
      |         en{4} = 'on';
      | end
      | set_param(gcb,'MaskVisibilities',en);
      mask Callback P_ext:
      | en = get_param(gcb,'MaskVisibilities');
      | 
      | switch get_param(gcb,'P_ext')
      |     case 'on'
      |         en{6} = 'off';
      |     case 'off'
      |         en{6} = 'on';
      | end
      | set_param(gcb,'MaskVisibilities',en);
      mask Display:
      | text(0.5,0.95,['{\bf Electric Source}'],'TexMode','on','horizontalAlignment', 'center')
      | text(0.5,0.1,['{(start)}'],'TexMode','on','horizontalAlignment', 'center')
      | 
      | port_label('input',1,'Source Current (A)')
      | port_label('input',2,'Source Voltage (V)')
      | 
      | port_label('output',1,'Source')
  Pump : Subsystem  mask(Liquid Pump){fld=Fuel, P_init=145, T_init=22, D=13*1e-3, L=0.1, rho=1000, cp=4, E=0, Omega_max=3000, DP_max=20, mdot_max=0.5, alpha=0.001}
      mask prompts: fld "Fluid Type"; P_init "Intial Outlet Pressure [kPa]"; T_init "Intial Outlet Temperature [°C]"; D "Pipe Internal Diameter [m]"; L "Pipe Length [m]"; rho "Fluid Density [kg/m^3]"; cp "Fluid Specific Heat [kJ/kgK]"; E "Fluid Modulus of Elasticity [N/m^2]"; Omega_max "Maximum Shaft Speed [RPM]"; DP_max "Maximum Pressure Difference [kPa]"; mdot_max "Maximum Mass Flow Rate [kg/s]"; alpha "Heat Generation Coefficient [kW/RPM]"
      mask help: Tracks the time rate of change of fluid temperature, mass flow rate, and power consumption.
      mask init:
      | load('Fluids.mat');
      | Fluid = eval(['Fluid.',fld]);
      settings: OpenFcn=|
      | load('Fluids.mat');
      | Set_Fluid_Popup_Names( Fluid )
      mask TypeOptions fld: Fuel | Water | Air | PG50
      mask DialogControl Container11 Prompt: Parameters
      mask DialogControl Container14 Prompt: Nonlinear Model
      mask DialogControl Container15 Prompt: Component Sizing - Nominal Values
      mask Display:
      | image(imread('centpump.jpg'))
      | 
      | text(0.5,0.95,['{\bf ',fld,' Pump}'],'TexMode','on','horizontalAlignment', 'center')
      | text(0.5,0.1,['{-----(P)}'],'TexMode','on','horizontalAlignment', 'center')
      | 
      | port_label('input',1,'Flow In')
      | port_label('input',2,'Power')
      | port_label('input',3,'Shaft Speed [RPM]')
      | port_label('output',1,'Flow Out')
  QLoad : Subsystem  mask{P_max=100, T0=20, eta_max=0.98, T_max=100, eta_min=0.8}
      mask prompts: P_max "Maximum Power [kW]"; T0 "Maximum Efficiency Temperature [oC]"; eta_max "Maximum Efficiency [0:1]"; T_max "Maximum Temperature [oC]"; eta_min "Minimum Efficiency [0:1]"
      mask init:
      | a = -(eta_max-eta_min)/(T_max-T0)^2;
      | b = -2*a*T0;
      | c = eta_max + a*T0^2;
      mask Display:
      | % text(0.5,0.9,['{\bf Load}'],'TexMode','on','horizontalAlignment', 'center')
      | 
      | port_label('input',1,'Power')
      | port_label('input',2,'Usage')
      | port_label('output',1,'Heat')
  Solenoid_P_to_M : Subsystem  mask(Solenoid (P to M)){fld=PG50, T_init=22, P_init=150, Tamb_init=22, f=0.05, KL=0, H=0, D=0.013, L=0.1, t=0.0015, E=2.4e6, v=0.4, e_rough=0.01*1e-3}
      mask prompts: fld "Fluid Type"; T_init "Initial Outlet Temperature [°C]"; P_init "Initial Outlet Pressure [kPa]"; Tamb_init "Initial Ambient Temperature [°C]"; f "Tube Friction Factor [-]"; KL "Minor Losses [-]"; H "Heat Transfer Coefficient [W/m²K]"; D "Internal Diameter [m]"; L "Length [m]"; t "Tube Wall Thickness [m]"; E "Tube Modulus of Elasticity [kPa]"; v "Tube Poisson Ratio [-]"; e_rough "Surface Roughness [m] (0.0015mm for copper, 0.01mm for rubber, 0mm for plastic)"
      mask help: Models an on/off solenoid given an upstream pressure and downstream mass flow rate.
      mask init:
      | load('Fluids.mat');
      | Fluid = eval(['Fluid.',fld]);
      | 
      | load('Moody.mat');
      settings: OpenFcn=|
      | load('Fluids.mat');
      | Set_Fluid_Popup_Names( Fluid )
      mask TypeOptions fld: Fuel | Water | Air | PG50
      mask DialogControl Container8 Prompt: Parameters
      mask DialogControl Container10 Prompt: Nonlinear Model
      mask DialogControl NomValuesGroupVar Prompt: Component Sizing - Nominal Values
      mask DialogControl Container11 Prompt: Linear Model
      mask Display:
      | image(imread('Solenoid.jpg'))
      | 
      | text(0.5,0.95,['{\bf ',fld,' Solenoid (P to M)}'],'TexMode','on','horizontalAlignment', 'center')
      | text(0.5,0.1,['{-----(P)}'],'TexMode','on','horizontalAlignment', 'center')
      | 
      | port_label('input',1,'Flow In')
      | port_label('input',2,'On/Off {1,0}')
      | port_label('output',1,'Flow Out')
  Solenoid_P_to_P : Subsystem  mask(Solenoid Valve (P to P)){fld=PG50, T_init=22, f=0.05, KL=0, D=0.013, L=0.1}
      mask prompts: fld "Fluid Type"; T_init "Initial Outlet Temperature [°C]"; f "Friction Factor [-]"; KL "Minor Losses [-]"; D "Internal Diameter [m]"; L "Length [m]"
      mask help: Models an on/off solenoid valve given upstream and downstream pressures.
      mask init:
      | load('Fluids.mat');
      | Fluid = eval(['Fluid.',fld]);
      | 
      | load('Moody.mat');
      settings: OpenFcn=|
      | load('Fluids.mat');
      | Set_Fluid_Popup_Names( Fluid )
      mask TypeOptions fld: Fuel | Water | Air | PG50
      mask DialogControl Container8 Prompt: Parameters
      mask DialogControl Container10 Prompt: Nonlinear Model
      mask DialogControl NomValuesGroupVar Prompt: Component Sizing - Nominal Values
      mask DialogControl Container11 Prompt: Linear Model
      mask Display:
      | image(imread('Solenoid.jpg'))
      | 
      | 
      | text(0.5,0.95,['{\bf ',fld,' Solenoid (P to P)}'],'TexMode','on','horizontalAlignment', 'center')
      | text(0.5,0.1,['{-----}'],'TexMode','on','horizontalAlignment', 'center')
      | 
      | port_label('input',1,'Flow In')
      | port_label('input',2,'On/Off {1,0}')
      | port_label('output',1,'Flow Out')
  Static Flow Junction : Subsystem  Commented=on  mask(Static Flow Junction){Num_In=2}
      mask prompts: Num_In "Number of Inlet Flows"
      mask help: Joins multiple flows into a single exit flow. Mass flow rates are taken from the upstream blocks. Note that the library link of the block is disabled when it is imported into a model.
      mask init:
      | h      = get_param(gcb,'handle');   % Get block handle
      | blk    = gcb; 
      | hblock = get(h);     % Parse out handles structure 
      | 
      | % delete any previous inports and bus selectors
      | for i = str2num(hblock.Num_In)+1:hblock.Ports(1)
      |     delete_block([blk,'/In',num2str(i)])
      |     delete_block([blk,'/b',num2str(i)])
      |     delete_block([blk,'/gm',num2str(i)])
      |     delete_block([blk,'/gt',num2str(i)])
      |     delete_block([blk,'/gp',num2str(i)])
      |     delete_block([blk,'/m',num2str(i)])
      |     delete_block([blk,'/p',num2str(i)])
      |     delete_block([blk,'/m2_',num2str(i)])
      |     delete_block([blk,'/t2_',num2str(i)])
      |     delete_block([blk,'/Divide',num2str(i)])
      |     
      | 	delete_unconnected_lines(blk)
      | end
      | 
      | % add the correct number of inputs to the add blocks
      | set_param([blk,'/Add'],'Inputs',char(repmat('+',1,str2num(hblock.Num_In))))
      | set_param([blk,'/Add1'],'Inputs',char(repmat('+',1,str2num(hblock.Num_In))))
      | set_param([blk,'/Add2'],'Inputs',char(repmat('+',1,str2num(hblock.Num_In))))
      | set_param([blk,'/Constant'],'Value',char(hblock.Num_In))
      | 
      | % generate inports, bus selectors, and route lines to each vector concat
      | for i = hblock.Ports(1)+1:str2num(hblock.Num_In)
      |     
      |     % add blocks
      |     add_block('simulink/Ports & Subsystems/In1',     [blk,'/In',num2str(i)],    'Position',[120 i*80-7 150 i*80+7]);         % adding inport   
      |     add_block([blk,'/b1'],                           [blk,'/b',num2str(i)],     'Position',[200 i*80-20+20-18 205 i*80-2+20+2]);         % adding inport
      |     add_block('simulink/Signal Routing/Goto',        [blk,'/gm',num2str(i)],    'Position',[260 i*80-17 340 i*80-3]);         % adding inport
      |     add_block('simulink/Signal Routing/Goto',        [blk,'/gt',num2str(i)],    'Position',[260 i*80+3 340 i*80+17]);         % adding inport
      |     add_block('simulink/Signal Routing/Goto',        [blk,'/gp',num2str(i)],    'Position',[260 i*80+6 340 i*80+20]);         % adding inport
      |     add_block('simulink/Signal Routing/From',        [blk,'/m',num2str(i)],     'Position',[410 i*80-20 490 i*80-2]);         % adding inport
      |     add_block('simulink/Signal Routing/From',        [blk,'/p',num2str(i)],     'Position',[1445 i*80-20 1525 i*80-2]);         % adding inport
      |     add_block('simulink/Signal Routing/From',        [blk,'/m2_',num2str(i)],   'Position',[730 i*80-20 810 i*80-2]);         % adding inport
      |     add_block('simulink/Signal Routing/From',        [blk,'/t2_',num2str(i)],   'Position',[730 i*80-20+24 810 i*80+24]);         % adding inport
      |     add_block([blk,'/Divide1'],                      [blk,'/Divide',num2str(i)],'Position',[825 i*80-20-7 841 i*80+27]);         % adding inport
      |     
      |     % set goto and from tags
      |     set_param([blk,'/gm',num2str(i)],'GotoTag',char(horzcat('m_in',num2str(i))))
      |     set_param([blk,'/gt',num2str(i)],'GotoTag',char(horzcat('T_in',num2str(i))))
      |     set_param([blk,'/gp',num2str(i)],'GotoTag',char(horzcat('P_in',num2str(i))))
      |     set_param([blk,'/m',num2str(i)],'GotoTag',char(horzcat('m_in',num2str(i))))
      |     set_param([blk,'/p',num2str(i)],'GotoTag',char(horzcat('P_in',num2str(i))))
      |     set_param([blk,'/m2_',num2str(i)],'GotoTag',char(horzcat('m_in',num2str(i))))
      |     set_param([blk,'/t2_',num2str(i)],'GotoTag',char(horzcat('T_in',num2str(i))))
      |    % set_param([blk,'/b',num2str(i)],'Outputs','3')
      |     
      |     % add lines
      |     add_line(blk,['In',num2str(i),'/1'], ['b',num2str(i),'/1'],'AutoRouting','on')
      |     add_line(blk,['b',num2str(i),'/1'],  ['gm',num2str(i),'/1'],'AutoRouting','on')
      |     add_line(blk,['b',num2str(i),'/2'],  ['gt',num2str(i),'/1'],'AutoRouting','on')
      |     add_line(blk,['b',num2str(i),'/3'],  ['gp',num2str(i),'/1'],'AutoRouting','on')
      |     add_line(blk,['m',num2str(i),'/1'],  ['Add/',num2str(i)],'AutoRouting','on')
      |     add_line(blk,['p',num2str(i),'/1'],  ['Add2/',num2str(i)],'AutoRouting','on')
      |     add_line(blk,['m2_',num2str(i),'/1'], ['Divide',num2str(i),'/1'],'AutoRouting','on')
      |     add_line(blk,['t2_',num2str(i),'/1'], ['Divide',num2str(i),'/2'],'AutoRouting','on')
      |     add_line(blk,['Divide',num2str(i),'/1'], ['Add1/',num2str(i)],'AutoRouting','on')
      |     
      |     % set goto and from background colors
      |     set_param([blk,'/gm',num2str(i)],'BackgroundColor','yellow') 
      |     set_param([blk,'/gt',num2str(i)],'BackgroundColor','yellow') 
      |     set_param([blk,'/gp',num2str(i)],'BackgroundColor','yellow') 
      |     set_param([blk,'/m',num2str(i)],'BackgroundColor','cyan') 
      |     set_param([blk,'/p',num2str(i)],'BackgroundColor','cyan') 
      |     set_param([blk,'/m2_',num2str(i)],'BackgroundColor','cyan') 
      |     set_param([blk,'/t2_',num2str(i)],'BackgroundColor','cyan') 
      |         
      | end
      settings: CopyFcn=|
      | h      = get_param(gcb,'handle');   % Get block handle
      | blk    = gcb;
      | 
      | set_param(blk, 'LinkStatus', 'inactive')
      mask Display:
      | image(fliplr(imread('Split.jpg')));
      | 
      | text(0.5,0.95,['{\bf Static Flow Junction}'],'TexMode','on','horizontalAlignment', 'center')
      | text(0.5,0.1,['{(X)}'],'TexMode','on','horizontalAlignment', 'center')
      | 
      | port_label('output',1,['Flow Out'])
      | 
      | h      = get_param(gcb,'handle');   % Get block handle
      | blk    = gcb;
      | hblock = get(h);     % Parse out handles structure
      | for i = 1:str2num(hblock.Num_In)
      |     port_label('input',i,horzcat('Flow In #',num2str(i)))
      | end
  Static Flow Split : Subsystem  Commented=on  mask(Static Flow Split){Num_Out=2}
      mask prompts: Num_Out "Number of Outlet Flows"
      mask help: Splits an inlet flow into multiple exit flows. Mass flow rates are taken from the downstream blocks. Note that the library link of the block is disabled when it is imported into a model.
      mask init:
      | h      = get_param(gcb,'handle');   % Get block handle
      | blk    = gcb; 
      | hblock = get(h);     % Parse out handles structure 
      | 
      | % delete any previous inports and bus selectors
      | for i = str2num(hblock.Num_Out)+1:hblock.Ports(2)
      |    delete_block([blk,'/Out',num2str(i)])
      |    delete_block([blk,'/m',num2str(i)])
      |    delete_block([blk,'/t',num2str(i)])
      |    delete_block([blk,'/p',num2str(i)])
      |    delete_block([blk,'/b',num2str(i)])
      |    delete_block([blk,'/Source',num2str(i)])
      |    delete_block([blk,'/g',num2str(i)])
      |    
      |    delete_unconnected_lines(blk)
      | end
      | 
      | % add the correct number of inputs to the add block
      | set_param([blk,'/Add'],'Inputs',char(repmat('+',1,str2num(hblock.Num_Out))))
      | 
      | % generate inports, bus selectors, and route lines to each vector concat
      | for i = hblock.Ports(2)+1:str2num(hblock.Num_Out)
      |     
      |     % add blocks
      |     add_block('simulink/Ports & Subsystems/Out1',   [blk,'/Out',num2str(i)],   'Position',[30 i*80-25+20 60 i*80-12+20]);         % adding inport
      |     add_block('simulink/Signal Routing/From',       [blk,'/m',num2str(i)],     'Position',[-150 i*80-20 -70 i*80-2]);         % adding inport
      |     add_block('simulink/Signal Routing/From',       [blk,'/t',num2str(i)],     'Position',[-150 i*80-20+20 -70 i*80-2+20]);         % adding inport
      |     add_block('simulink/Signal Routing/From',       [blk,'/p',num2str(i)],     'Position',[-150 i*80-20+40 -70 i*80-2+40]);         % adding inport
      |     add_block('simulink/Signal Routing/Bus Creator',[blk,'/b',num2str(i)],     'Position',[5 i*80-20+20-18 10 i*80-2+20+2]);         % adding inport
      |     add_block('DAEMOT_Lib/Support Functions/Source',[blk,'/Source',num2str(i)],'Position',[395 i*80-14 460 i*80+14]);         % adding inport
      |     add_block('simulink/Signal Routing/Goto',       [blk,'/g',num2str(i)],     'Position',[505 i*80-9 585 i*80+9]);         % adding inport
      |     
      |     % set goto and from tags
      |     set_param([blk,'/m',num2str(i)],'GotoTag',char(horzcat('m_dot',num2str(i))))
      |     set_param([blk,'/t',num2str(i)],'GotoTag',char('T_in'))
      |     set_param([blk,'/p',num2str(i)],'GotoTag',char('P_in'))
      |     set_param([blk,'/g',num2str(i)],'GotoTag',char(['m_dot',num2str(i)]))
      |     set_param([blk,'/b',num2str(i)],'Inputs','3')
      |     
      |     % set goto and from background colors
      |     set_param([blk,'/t',num2str(i)],'BackgroundColor','cyan')
      |     set_param([blk,'/m',num2str(i)],'BackgroundColor','cyan') 
      |     set_param([blk,'/p',num2str(i)],'BackgroundColor','cyan') 
      |     set_param([blk,'/g',num2str(i)],'BackgroundColor','yellow')    
      |     
      |     % add lines
      |     add_line(blk,['m',num2str(i),'/1'],['b',num2str(i),'/1'],'AutoRouting','on')
      |     add_line(blk,['t',num2str(i),'/1'],['b',num2str(i),'/2'],'AutoRouting','on')
      |     add_line(blk,['p',num2str(i),'/1'],['b',num2str(i),'/3'],'AutoRouting','on')
      |     add_line(blk,['b',num2str(i),'/1'],['Out',num2str(i),'/1'],'AutoRouting','on')
      |     add_line(blk,['Source',num2str(i),'/1'],['g',num2str(i),'/1'],'AutoRouting','on')
      |     add_line(blk,['Source',num2str(i),'/1'],['Add/',num2str(i)],'AutoRouting','on')
      |     
      |     % set line names for mass flow bus
      |     p = get_param([blk,'/m',num2str(i)], 'PortHandles');
      |     l = get_param(p.Outport,'Line');
      |     set_param(l,'Name','mdot_kgps')
      |     
      |     % set line names for temperature bus
      |     p = get_param([blk,'/t',num2str(i)], 'PortHandles');
      |     l = get_param(p.Outport,'Line');
      |     set_param(l,'Name','T_C')
      |     
      |     % set line names for pressure bus
      |     p = get_param([blk,'/p',num2str(i)], 'PortHandles');
      |     l = get_param(p.Outport,'Line');
      |     set_param(l,'Name','P_kPa')
      | end
      | 
      | clear h blk hblock
      settings: CopyFcn=|
      | h      = get_param(gcb,'handle');   % Get block handle
      | blk    = gcb;
      | 
      | set_param(blk, 'LinkStatus', 'inactive')
      mask Display:
      | image(imread('Split.jpg'));
      | 
      | text(0.5,0.95,['{\bf Static Flow Split}'],'TexMode','on','horizontalAlignment', 'center')
      | text(0.5,0.1,['{(X)}'],'TexMode','on','horizontalAlignment', 'center')
      | 
      | port_label('input',1,['Flow In'])
      | 
      | h      = get_param(gcb,'handle');   % Get block handle
      | blk    = gcb;
      | hblock = get(h);     % Parse out handles structure
      | for i = 1:str2num(hblock.Num_Out)
      |     port_label('output',i,horzcat('Flow Out #',num2str(i)))
      | end
  Switch : Subsystem  mask(Switch){}
      mask help: This is a switch.
  To LabVIEW_Old : Subsystem  Commented=on
  Two_Way_Valve_P_to_P : Subsystem  mask(Two Way Valve (P to P)){fld=PG50, T_init=22, f=0.05, KL=0, D=0.013, L=0.1}
      mask prompts: fld "Fluid Type"; T_init "Initial Outlet Temperature [°C]"; f "Friction Factor [-]"; KL "Minor Losses [-]"; D "Internal Diameter [m]"; L "Length [m]"
      mask help: Models a two-way variable valve given upstream and downstream pressures.
      mask init:
      | load('Fluids.mat');
      | Fluid = eval(['Fluid.',fld]);
      | 
      | load('Moody.mat');
      settings: OpenFcn=|
      | load('Fluids.mat');
      | Set_Fluid_Popup_Names( Fluid )
      mask TypeOptions fld: Fuel | Water | Air | PG50
      mask DialogControl Container8 Prompt: Parameters
      mask DialogControl Container10 Prompt: Nonlinear Model
      mask DialogControl NomValuesGroupVar Prompt: Component Sizing - Nominal Values
      mask DialogControl Container11 Prompt: Linear Model
      mask Display:
      | image(imread('Solenoid.jpg'))
      | 
      | 
      | text(0.5,0.95,['{\bf ',fld,' Continuous Valve (P to P)}'],'TexMode','on','horizontalAlignment', 'center')
      | text(0.5,0.1,['{-----}'],'TexMode','on','horizontalAlignment', 'center')
      | 
      | port_label('input',1,'Flow In')
      | port_label('input',2,'Fraction of Flow 1 [0,1]')
      | port_label('output',1,'Flow Out 1')
      | port_label('output',2,'Flow Out 2')
  UDP_Controller_SR_old : Subsystem  Commented=on  mask(Send/Receive to UDP Controller){conn=1, update_rate=1, in_size=1, out_size=1, port_in=61176, loc_port_in=61177, port_out=61166, loc_port_out=61167}
      mask prompts: conn "Connection Number [1-10]"; update_rate "Controller Update Rate (s)"; in_size "Controller Input Size"; out_size "Controller Output Size"; port_in "Input Port"; loc_port_in "Input Local Port"; port_out "Output Port"; loc_port_out "Output Local Port"
      mask help: Sends and retrieves data from a controller over a UDP connection. Passes data over UDP at 10 Hz but applies a sample and hold at the update rate of the controller.
      mask init:
      | block = gcb;
      | 
      | port_in     = '61576';
      | loc_port_in = '61577';
      | 
      | port_out     = '61566';
      | loc_port_out = '61567';
      | 
      | port_in      = [port_in(1:2)     ,conn,port_in(4:5)];
      | loc_port_in  = [loc_port_in(1:2) ,conn,loc_port_in(4:5)];
      | port_out     = [port_out(1:2)    ,conn,port_out(4:5)];
      | loc_port_out = [loc_port_out(1:2),conn,loc_port_out(4:5)];
      | 
      | set_param(gcb,'port_in'     ,port_in);
      | set_param(gcb,'loc_port_in' ,loc_port_in);
      | set_param(gcb,'port_out'    ,port_out);
      | set_param(gcb,'loc_port_out',loc_port_out);
      | 
      | set_param([gcb,'/To Controller/UDP Send'],'Port',port_in);
      | set_param([gcb,'/To Controller/UDP Send'],'LocalPort',loc_port_in);
      | 
      | set_param([gcb,'/From Controller/MEASUREMENTS1/UDP Receive'],'Port',port_out);
      | set_param([gcb,'/From Controller/MEASUREMENTS1/UDP Receive'],'LocalPort',loc_port_out);
      mask Display: disp(['Send/Receive to UDP Controller\n\nConnection: ',conn,'\n\nUpdate Rate (s): ',num2str(update_rate),'s\n\nInput Size: ',num2str(in_size),'\n\nOutput Size: ',num2str(out_size)])
  UDP_Controller_old : Subsystem  Commented=on  mask{ctrl_fcn=Ctrl_Fcn(u), conn=1, update_rate=1, in_size=1, out_size=1, port_in=61177, loc_port_in=61176, port_out=61167, loc_port_out=61166}
      mask prompts: ctrl_fcn "Controller Function Name"; conn "Connection Number [1-10]"; update_rate "Controller Update Rate (s)"; in_size "Controller Input Size"; out_size "Controller Output Size"; port_in "Input Port"; loc_port_in "Input Local Port"; port_out "Output Port"; loc_port_out "Output Local Port"
      mask help: Solves a controller with inputs/outputs sent over a UDP connection. The UDP Receive sample time is set to the controller update rate.
      mask init:
      | block = gcb;
      | 
      | port_in     = '61577';
      | loc_port_in = '61576';
      | 
      | port_out     = '61567';
      | loc_port_out = '61566';
      | 
      | port_in      = [port_in(1:2)     ,conn,port_in(4:5)];
      | loc_port_in  = [loc_port_in(1:2) ,conn,loc_port_in(4:5)];
      | port_out     = [port_out(1:2)    ,conn,port_out(4:5)];
      | loc_port_out = [loc_port_out(1:2),conn,loc_port_out(4:5)];
      | 
      | set_param(gcb,'port_in'     ,port_in);
      | set_param(gcb,'loc_port_in' ,loc_port_in);
      | set_param(gcb,'port_out'    ,port_out);
      | set_param(gcb,'loc_port_out',loc_port_out);
      | 
      | set_param([gcb,'/Controller'],'MATLABFcn',ctrl_fcn);
      | 
      | set_param([gcb,'/To Controller/UDP Receive'],'Port',port_in);
      | set_param([gcb,'/To Controller/UDP Receive'],'LocalPort',loc_port_in);
      | set_param([gcb,'/To Controller/UDP Receive'],'SampleTime',num2str(update_rate));
      | set_param([gcb,'/To Controller/UDP Receive'],'Timeout',num2str(update_rate+5));
      | 
      | set_param([gcb,'/From Controller'],'SystemSampleTime',num2str(update_rate));
      | set_param([gcb,'/From Controller/UDP Send'],'Port',port_out);
      | set_param([gcb,'/From Controller/UDP Send'],'LocalPort',loc_port_out);
      | 
      | set_param(bdroot,'FixedStep',num2str(update_rate))
      mask Display: disp(['UDP Controller\n\nFunction: ',ctrl_fcn,'\n\nConnection: ',conn,'\n\nUpdate Rate (s): ',num2str(update_rate),'s\n\nInput Size: ',num2str(in_size),'\n\nOutput Size: ',num2str(out_size)])
  Upper to Lower Edge Preview_old : Subsystem  Commented=on  SystemSampleTime=dt_l  mask{hor_u=5, dt_u=10, hor_l=5, dt_l=1}
      mask prompts: hor_u "Upper Level Horizon"; dt_u "Upper Level Timestep"; hor_l "Lower Level Horizon"; dt_l "Lower Level Timestep"
  Wall : Subsystem  mask(Wall){Num_Out=1, Tw_init=20, M_wall=1, Cp_wall=0.9}
      mask prompts: Num_Out "Number of Fluid Flows"; Tw_init "Initial Wall Temperature [°C]"; M_wall "Wall Mass [kg]"; Cp_wall "Wall Specific Heat [kJ/kg*K]"
      mask help: Tracks the time rate of change of wall temperature based on convective heat transfer calculated downstream.
      mask init:
      | h      = get_param(gcb,'handle');   % Get block handle
      | blk    = gcb;
      | hblock = get(h);     % Parse out handles structure
      | 
      | % delete any previous inports and bus selectors
      | for i = str2num(hblock.Num_Out)+1:hblock.Ports(2)
      |     delete_block([blk,'/s',num2str(i)])
      |     delete_block([blk,'/g',num2str(i)])
      |     %delete_block([blk,'/f',num2str(i)])
      |     delete_block([blk,'/b',num2str(i)])
      |     delete_block([blk,'/o',num2str(i)])
      |     delete_block([blk,'/h',num2str(i)])
      | end
      | delete_unconnected_lines(blk)
      | 
      | set_param([blk,'/Mux_In_2'],'Inputs',num2str(hblock.Num_Out))
      | 
      | for i = hblock.Ports(2)+1:str2num(hblock.Num_Out)
      |     add_block([blk,'/s1'],[blk,'/s',num2str(i)],'Position',[200 i*80-20+20-18 205 i*80-2+20+2]);         % adding inport
      |     add_block([blk,'/g1'],[blk,'/g',num2str(i)],'Position',[200 i*80-20+20-18 205 i*80-2+20+2]);         % adding inport
      |     %add_block([blk,'/f1'],[blk,'/f',num2str(i)],'Position',[200 i*80-20+20-18 205 i*80-2+20+2]);         % adding inport
      |     add_block([blk,'/b1'],[blk,'/b',num2str(i)],'Position',[200 i*80-20+20-18 205 i*80-2+20+2]);         % adding inport
      |     add_block([blk,'/o1'],[blk,'/o',num2str(i)],'Position',[200 i*80-20+20-18 205 i*80-2+20+2]);         % adding inport
      |     add_block([blk,'/h1'],[blk,'/h',num2str(i)],'Position',[200 i*80-20+20-18 205 i*80-2+20+2]);         % adding inport
      |     
      |     set_param([blk,'/g',num2str(i)],'GotoTag',char(horzcat('Q_fluid',num2str(i))))
      |     set_param([blk,'/h',num2str(i)],'GotoTag',char(horzcat('Q_fluid',num2str(i))))
      | 
      |     % add lines
      |     add_line(blk,['s',num2str(i),'/1'], ['g',num2str(i),'/1'],'AutoRouting','on')
      |     add_line(blk,['f1','/1'], ['b',num2str(i),'/1'],'AutoRouting','on')
      |     add_line(blk,['b',num2str(i),'/1'], ['o',num2str(i),'/1'],'AutoRouting','on')
      |     
      |     add_line(blk,['h',num2str(i),'/1'], ['Mux_In_2/',num2str(i)],'AutoRouting','on')
      | end
      | 
      | 
      | 
      | clear h blk hblock
      settings: OpenFcn=|
      | load('Fluids.mat');
      | Set_Fluid_Popup_Names( Fluid )
      mask DialogControl Container5 Prompt: Parameters
      mask DialogControl Container8 Prompt: Nonlinear Model
      mask DialogControl Container13 Prompt: Component Sizing - Nominal Values
      mask DialogControl Container11 Prompt: Linear Model
      mask Display:
      | image(imread('ColdPlate.jpg'))
      | 
      | text(0.5,0.95,['{\bfWall}'],'TexMode','on','horizontalAlignment', 'center')
      | text(0.5,0.08,['{(T)}'],'TexMode','on','horizontalAlignment', 'center')
      | 
      | port_label('input',1,'Heat Load [kW]')
      | 
      | for i = 1:Num_Out
      |     port_label('output',i,horzcat('Flow #',num2str(i)))
      | end
